simulink model "FOC_sensored"  (R2026a)
settings: Solver=VariableStepAuto  StopTime=0.5  MaxStep=1e-4  RelTol=1e-4
values from neighbouring files (symbols this model uses):
  Encoder_resolution = 4000    [FOC_sensored_script.m]
  In = 1    [FOC_sensored_script.m]
  J = 0.1e-4    (= 1e-05)    [FOC_sensored_script.m]
  Kr_cont_current = (2*omega_n*tau_q*zeta - 1) / K_q    [FOC_sensored_script.m]
  Kr_cont_speed = (2*omega_n_speed*tau_w*zeta_speed - 1) / K_w    [FOC_sensored_script.m]
  Kr_direct_back_current = (1-delta2*exp(Ts_current/tau_q)) / (K_q*(exp(Ts_current/tau_q)-1))    [FOC_sensored_script.m]
  Kr_direct_back_speed = (1-delta2*exp(Ts_speed/tau_w)) / (K_w*(exp(Ts_speed/tau_w)-1))    [FOC_sensored_script.m]
  Kr_direct_forw_current = (1+(1+delta1)*exp(Ts_current/tau_q)) / (K_q*(exp(Ts_current/tau_q)-1))    [FOC_sensored_script.m]
  Kr_direct_tustin_current = (2-exp(Ts_current/tau_q)*(delta2-delta1-1)) / (2*K_q*(exp(Ts_current/tau_q)-1))    [FOC_sensored_script.m]
  Kr_direct_tustin_speed = (2-exp(Ts_speed/tau_w)*(delta2-delta1-1)) / (2*K_w*(exp(Ts_speed/tau_w)-1))    [FOC_sensored_script.m]
  Ls = 330e-6/2    (= 0.000165)    [FOC_sensored_script.m]
  Mn = Pn/wn    [FOC_sensored_script.m]
  nn = ns/pp    (= 6000)    [FOC_sensored_script.m]
  pp = (60*fs)/ns    (= 4)    [FOC_sensored_script.m]
  Psir = 0.0064    [FOC_sensored_script.m]
  T_speed_feedback = 0.0005    [FOC_sensored_script.m]
  Ti_cont_current = (2*omega_n*tau_q*zeta - 1) / (tau_q * omega_n^2)    [FOC_sensored_script.m]
  Ti_cont_speed = (2*omega_n_speed*tau_w*zeta_speed - 1) / (tau_w * omega_n_speed^2)    [FOC_sensored_script.m]
  Ti_direct_back_current = Ts_current * (exp(-Ts_current/tau_q)-delta2) / (1+delta1+delta2)    [FOC_sensored_script.m]
  Ti_direct_back_speed = Ts_speed * (exp(-Ts_speed/tau_w)-delta2) / (1+delta1+delta2)    [FOC_sensored_script.m]
  Ti_direct_forw_current = Ts_current * (1+delta1+exp(-Ts_current/tau_q)) / (1+delta1+delta2)    [FOC_sensored_script.m]
  Ti_direct_forw_speed = Ts_speed * (1+delta1+exp(-Ts_speed/tau_w)) / (1+delta1+delta2)    [FOC_sensored_script.m]
  Ti_direct_tustin_current = Ts_current*(2*exp(-Ts_current/tau_q)+delta1-delta2+1) / (2*(1+delta1+delta2))    [FOC_sensored_script.m]
  Ti_direct_tustin_speed = Ts_speed*(2*exp(-Ts_speed/tau_w)+delta1-delta2+1) / (2*(1+delta1+delta2))    [FOC_sensored_script.m]
  Ts_current = 100e-6    (= 0.0001)    [FOC_sensored_script.m]
  Udc = 24    [FOC_sensored_script.m]
undefined symbols (not defined in the file or in its folder): Ld, Lq
libraries: fl_lib x48, nesl_utility x42, ee_lib x18, eeTransforms x12
(part 1 of 3)
settings Model: Creator=LukaPravica  LastModifiedBy=Rio
settings SimscapeCC: ExplicitSolverDiagnosticOptions=none  SimscapeNominalValues="[{\"value\":\"1\",\"unit\":\"A\"},{\"value\":\"1\",\"unit\":\"bar\"},{\"value\":\"1\",\"unit\":\"cm^2\"},{\"value\":\"1\",\"unit\":\"cm^3/s\"},{\"value\":\"1\",\"unit\":\"kJ/kg\"},{\"value\":\"1\",\"unit\":\"kW\"},{\"value\":\"1\",\"unit\":\"l\"},{\"value\":\"1\",\"unit\":\"N\"},{\"value\":\"1\",\"unit\":\"N*m\"},{\"value\":\"1\",\"unit\":\"V\"}]"  SimscapeLogType=none  SimscapeLogDataHistory=5000.0

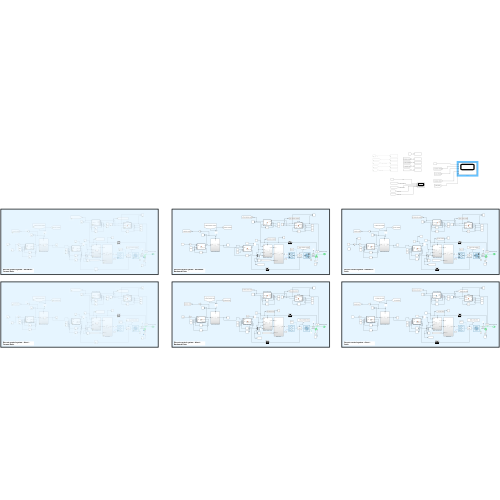
[thumbnail: Simulink's stored preview of the top-level diagram]
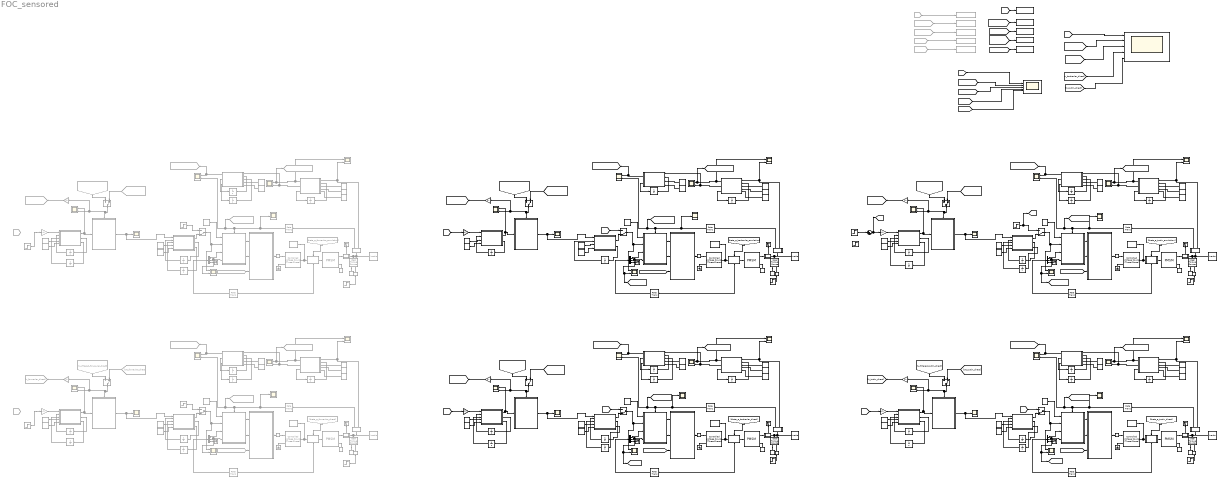
== system FOC_sensored ==
  note: Discrete control system - emulation - Tustin
  note: Discrete control system - direct - Tustin
  note: Discrete control system - emulation -
      | Backward Euler
  note: Discrete control system - direct - Backward Euler
  note: Discrete control system - emulation -
      | Forward Euler
  note: Discrete control system - direct -
      | Forward Euler
  Constant{,1,20,30} (4 alike) : Constant  Value=0  SampleTime=Ts_current
  Constant{3,5,8,10..11,13,15,18,21,23,25,28,31,33,35,38} (16 alike) : Constant  Value=Ts_current  SampleTime=Ts_current
  Constant{2,12,22,32} (4 alike) : Constant  Value=1/(2*pi*T_speed_feedback)  SampleTime=Ts_current
  Constant{4,14,24,34} (4 alike) : Constant  Value=Encoder_resolution  SampleTime=Ts_current
  Constant{6,16,26,36} (4 alike) : Constant  Value=pp  SampleTime=Ts_current
  Constant17 : Constant  Value=1/(2*pi*Ti_direct_tustin_current)  SampleTime=Ts_current
  Constant19 : Constant  Value=1/(2*pi*Ti_direct_tustin_speed)  SampleTime=Ts_current
  Constant27 : Constant  Value=1/(2*pi*Ti_cont_current)  SampleTime=Ts_current
  Constant29 : Constant  Value=1/(2*pi*Ti_cont_speed)  SampleTime=Ts_current
  Constant37 : Constant  Value=1/(2*pi*Ti_direct_back_current)  SampleTime=Ts_current
  Constant39 : Constant  Value=1/(2*pi*Ti_direct_back_speed)  SampleTime=Ts_current
  Constant40 : Constant  Commented=on  Value=0  SampleTime=Ts_current
  Constant{41,43,45,48,51,53,55,58} (8 alike) : Constant  Commented=on  Value=Ts_current  SampleTime=Ts_current
  Constant42 : Constant  Commented=on  Value=1/(2*pi*T_speed_feedback)  SampleTime=Ts_current
  Constant44 : Constant  Commented=on  Value=Encoder_resolution  SampleTime=Ts_current
  Constant46 : Constant  Commented=on  Value=pp  SampleTime=Ts_current
  Constant47 : Constant  Commented=on  Value=1/(2*pi*Ti_cont_current)  SampleTime=Ts_current
  Constant49 : Constant  Commented=on  Value=1/(2*pi*Ti_cont_speed)  SampleTime=Ts_current
  Constant50 : Constant  Commented=on  Value=0  SampleTime=Ts_current
  Constant52 : Constant  Commented=on  Value=1/(2*pi*T_speed_feedback)  SampleTime=Ts_current
  Constant54 : Constant  Commented=on  Value=Encoder_resolution  SampleTime=Ts_current
  Constant56 : Constant  Commented=on  Value=pp  SampleTime=Ts_current
  Constant57 : Constant  Commented=on  Value=1/(2*pi*Ti_direct_forw_current)  SampleTime=Ts_current
  Constant59 : Constant  Commented=on  Value=1/(2*pi*Ti_direct_forw_speed)  SampleTime=Ts_current
  Constant7 : Constant  Value=1/(2*pi*Ti_cont_current)  SampleTime=Ts_current
  Constant9 : Constant  Value=1/(2*pi*Ti_cont_speed)  SampleTime=Ts_current
  Controlled Voltage Source (Three-Phase){1,3..4,7} (4 alike) : ee_lib/Sources/Controlled Voltage Source (Three-Phase)  input_option=ee.enum.inputType.instantaneous  FRated=60 Hz
  Controlled Voltage Source (Three-Phase)2 : ee_lib/Sources/Controlled Voltage Source (Three-Phase)  Commented=on  input_option=ee.enum.inputType.instantaneous  FRated=60 Hz
  Controlled Voltage Source (Three-Phase)5 : ee_lib/Sources/Controlled Voltage Source (Three-Phase)  Commented=on  input_option=ee.enum.inputType.instantaneous  FRated=60 Hz
  Demux{1,3..4,7} (4 alike) : Demux  Outputs=3
  Demux2 : Demux  Commented=on  Outputs=3
  Demux5 : Demux  Commented=on  Outputs=3
  Diskretni regulator brzine1 : Subsystem
      settings: PortSchema="{\"entries\":[{\"content\":{\"sides\":[{\"content\":{\"connectorIds\":[\"In1\"]},\"type\":\"ConnectorPlacement.EquallySpacedRectSide\",\"uuid\":\"a9765fbc-5a4d-474e-be8d-5c320c5f07ca\"},{\"content\":{\"connectorIds\":[\"Out1\"],\"side\":\"RIGHT\"},\"type\":\"ConnectorPlacement.EquallySpacedRectSide\",\"uuid\":\"d113e0d0-4772-4877-8676-69342ee8f64f\"},{\"content\":{\"connectorIds\":[\"In2\"],\"side\":\"TOP\"},\"type\":\"ConnectorPlacement.EquallySpacedRectSide\",\"uuid\":\"4ca0dc59-fd41-4846-82a7-6904cf53659d\"}]},\"type\":\"ConnectorPlacement.EquallySpacedConnector\",\"uuid\":\"7fdfac1a-ebdc-43ed-9adb-be729266989d\"}],\"packageUris\":[\"http://schema.mathworks.com/mf0/Connector/R2020b\"],\"version\":\"1.0\"}"
  Diskretni regulator brzine2 : Subsystem
      settings: PortSchema="{\"entries\":[{\"content\":{\"sides\":[{\"content\":{\"connectorIds\":[\"In1\"]},\"type\":\"ConnectorPlacement.EquallySpacedRectSide\",\"uuid\":\"a9765fbc-5a4d-474e-be8d-5c320c5f07ca\"},{\"content\":{\"connectorIds\":[\"Out1\"],\"side\":\"RIGHT\"},\"type\":\"ConnectorPlacement.EquallySpacedRectSide\",\"uuid\":\"d113e0d0-4772-4877-8676-69342ee8f64f\"},{\"content\":{\"connectorIds\":[\"In2\"],\"side\":\"TOP\"},\"type\":\"ConnectorPlacement.EquallySpacedRectSide\",\"uuid\":\"4ca0dc59-fd41-4846-82a7-6904cf53659d\"}]},\"type\":\"ConnectorPlacement.EquallySpacedConnector\",\"uuid\":\"7fdfac1a-ebdc-43ed-9adb-be729266989d\"}],\"packageUris\":[\"http://schema.mathworks.com/mf0/Connector/R2020b\"],\"version\":\"1.0\"}"
  Diskretni regulator brzine3 : Subsystem
      settings: PortSchema="{\"entries\":[{\"content\":{\"sides\":[{\"content\":{\"connectorIds\":[\"In1\"]},\"type\":\"ConnectorPlacement.EquallySpacedRectSide\",\"uuid\":\"a9765fbc-5a4d-474e-be8d-5c320c5f07ca\"},{\"content\":{\"connectorIds\":[\"Out1\"],\"side\":\"RIGHT\"},\"type\":\"ConnectorPlacement.EquallySpacedRectSide\",\"uuid\":\"d113e0d0-4772-4877-8676-69342ee8f64f\"},{\"content\":{\"connectorIds\":[\"In2\"],\"side\":\"TOP\"},\"type\":\"ConnectorPlacement.EquallySpacedRectSide\",\"uuid\":\"4ca0dc59-fd41-4846-82a7-6904cf53659d\"}]},\"type\":\"ConnectorPlacement.EquallySpacedConnector\",\"uuid\":\"7fdfac1a-ebdc-43ed-9adb-be729266989d\"}],\"packageUris\":[\"http://schema.mathworks.com/mf0/Connector/R2020b\"],\"version\":\"1.0\"}"
  Diskretni regulator brzine4 : Subsystem  Commented=on
      settings: PortSchema="{\"entries\":[{\"content\":{\"sides\":[{\"content\":{\"connectorIds\":[\"In1\"]},\"type\":\"ConnectorPlacement.EquallySpacedRectSide\",\"uuid\":\"a9765fbc-5a4d-474e-be8d-5c320c5f07ca\"},{\"content\":{\"connectorIds\":[\"Out1\"],\"side\":\"RIGHT\"},\"type\":\"ConnectorPlacement.EquallySpacedRectSide\",\"uuid\":\"d113e0d0-4772-4877-8676-69342ee8f64f\"},{\"content\":{\"connectorIds\":[\"In2\"],\"side\":\"TOP\"},\"type\":\"ConnectorPlacement.EquallySpacedRectSide\",\"uuid\":\"4ca0dc59-fd41-4846-82a7-6904cf53659d\"}]},\"type\":\"ConnectorPlacement.EquallySpacedConnector\",\"uuid\":\"7fdfac1a-ebdc-43ed-9adb-be729266989d\"}],\"packageUris\":[\"http://schema.mathworks.com/mf0/Connector/R2020b\"],\"version\":\"1.0\"}"
  Diskretni regulator brzine5 : Subsystem
      settings: PortSchema="{\"entries\":[{\"content\":{\"sides\":[{\"content\":{\"connectorIds\":[\"In1\"]},\"type\":\"ConnectorPlacement.EquallySpacedRectSide\",\"uuid\":\"a9765fbc-5a4d-474e-be8d-5c320c5f07ca\"},{\"content\":{\"connectorIds\":[\"Out1\"],\"side\":\"RIGHT\"},\"type\":\"ConnectorPlacement.EquallySpacedRectSide\",\"uuid\":\"d113e0d0-4772-4877-8676-69342ee8f64f\"},{\"content\":{\"connectorIds\":[\"In2\"],\"side\":\"TOP\"},\"type\":\"ConnectorPlacement.EquallySpacedRectSide\",\"uuid\":\"4ca0dc59-fd41-4846-82a7-6904cf53659d\"}]},\"type\":\"ConnectorPlacement.EquallySpacedConnector\",\"uuid\":\"7fdfac1a-ebdc-43ed-9adb-be729266989d\"}],\"packageUris\":[\"http://schema.mathworks.com/mf0/Connector/R2020b\"],\"version\":\"1.0\"}"
  Diskretni regulator brzine6 : Subsystem  Commented=on
      settings: PortSchema="{\"entries\":[{\"content\":{\"sides\":[{\"content\":{\"connectorIds\":[\"In1\"]},\"type\":\"ConnectorPlacement.EquallySpacedRectSide\",\"uuid\":\"a9765fbc-5a4d-474e-be8d-5c320c5f07ca\"},{\"content\":{\"connectorIds\":[\"Out1\"],\"side\":\"RIGHT\"},\"type\":\"ConnectorPlacement.EquallySpacedRectSide\",\"uuid\":\"d113e0d0-4772-4877-8676-69342ee8f64f\"},{\"content\":{\"connectorIds\":[\"In2\"],\"side\":\"TOP\"},\"type\":\"ConnectorPlacement.EquallySpacedRectSide\",\"uuid\":\"4ca0dc59-fd41-4846-82a7-6904cf53659d\"}]},\"type\":\"ConnectorPlacement.EquallySpacedConnector\",\"uuid\":\"7fdfac1a-ebdc-43ed-9adb-be729266989d\"}],\"packageUris\":[\"http://schema.mathworks.com/mf0/Connector/R2020b\"],\"version\":\"1.0\"}"
  Diskretni regulatori struje1 : Subsystem
      settings: PortSchema="{\"entries\":[{\"content\":{\"sides\":[{\"content\":{\"connectorIds\":[\"In1\",\"In2\",\"In3\",\"In4\"]},\"type\":\"ConnectorPlacement.EquallySpacedRectSide\",\"uuid\":\"d3a62493-f7c6-444f-9476-25937989f6ea\"},{\"content\":{\"connectorIds\":[\"Out1\",\"Out2\"],\"side\":\"RIGHT\"},\"type\":\"ConnectorPlacement.EquallySpacedRectSide\",\"uuid\":\"ca5c9823-b9be-4b72-ab87-a2cad855a0f6\"},{\"content\":{\"connectorIds\":[\"In5\"],\"side\":\"TOP\"},\"type\":\"ConnectorPlacement.EquallySpacedRectSide\",\"uuid\":\"496b345e-fed9-4adb-95d9-010d07f11d94\"}]},\"type\":\"ConnectorPlacement.EquallySpacedConnector\",\"uuid\":\"9eb14200-6fae-48ad-9447-ab4bb77ea536\"}],\"packageUris\":[\"http://schema.mathworks.com/mf0/Connector/R2020b\"],\"version\":\"1.0\"}"
  Diskretni regulatori struje2 : Subsystem
      settings: PortSchema="{\"entries\":[{\"content\":{\"sides\":[{\"content\":{\"connectorIds\":[\"In1\",\"In2\",\"In3\",\"In4\"]},\"type\":\"ConnectorPlacement.EquallySpacedRectSide\",\"uuid\":\"d3a62493-f7c6-444f-9476-25937989f6ea\"},{\"content\":{\"connectorIds\":[\"Out1\",\"Out2\"],\"side\":\"RIGHT\"},\"type\":\"ConnectorPlacement.EquallySpacedRectSide\",\"uuid\":\"ca5c9823-b9be-4b72-ab87-a2cad855a0f6\"},{\"content\":{\"connectorIds\":[\"In5\"],\"side\":\"TOP\"},\"type\":\"ConnectorPlacement.EquallySpacedRectSide\",\"uuid\":\"496b345e-fed9-4adb-95d9-010d07f11d94\"}]},\"type\":\"ConnectorPlacement.EquallySpacedConnector\",\"uuid\":\"9eb14200-6fae-48ad-9447-ab4bb77ea536\"}],\"packageUris\":[\"http://schema.mathworks.com/mf0/Connector/R2020b\"],\"version\":\"1.0\"}"
  Diskretni regulatori struje3 : Subsystem
      settings: PortSchema="{\"entries\":[{\"content\":{\"sides\":[{\"content\":{\"connectorIds\":[\"In1\",\"In2\",\"In3\",\"In4\"]},\"type\":\"ConnectorPlacement.EquallySpacedRectSide\",\"uuid\":\"d3a62493-f7c6-444f-9476-25937989f6ea\"},{\"content\":{\"connectorIds\":[\"Out1\",\"Out2\"],\"side\":\"RIGHT\"},\"type\":\"ConnectorPlacement.EquallySpacedRectSide\",\"uuid\":\"ca5c9823-b9be-4b72-ab87-a2cad855a0f6\"},{\"content\":{\"connectorIds\":[\"In5\"],\"side\":\"TOP\"},\"type\":\"ConnectorPlacement.EquallySpacedRectSide\",\"uuid\":\"496b345e-fed9-4adb-95d9-010d07f11d94\"}]},\"type\":\"ConnectorPlacement.EquallySpacedConnector\",\"uuid\":\"9eb14200-6fae-48ad-9447-ab4bb77ea536\"}],\"packageUris\":[\"http://schema.mathworks.com/mf0/Connector/R2020b\"],\"version\":\"1.0\"}"
  Diskretni regulatori struje4 : Subsystem  Commented=on
      settings: PortSchema="{\"entries\":[{\"content\":{\"sides\":[{\"content\":{\"connectorIds\":[\"In1\",\"In2\",\"In3\",\"In4\"]},\"type\":\"ConnectorPlacement.EquallySpacedRectSide\",\"uuid\":\"d3a62493-f7c6-444f-9476-25937989f6ea\"},{\"content\":{\"connectorIds\":[\"Out1\",\"Out2\"],\"side\":\"RIGHT\"},\"type\":\"ConnectorPlacement.EquallySpacedRectSide\",\"uuid\":\"ca5c9823-b9be-4b72-ab87-a2cad855a0f6\"},{\"content\":{\"connectorIds\":[\"In5\"],\"side\":\"TOP\"},\"type\":\"ConnectorPlacement.EquallySpacedRectSide\",\"uuid\":\"496b345e-fed9-4adb-95d9-010d07f11d94\"}]},\"type\":\"ConnectorPlacement.EquallySpacedConnector\",\"uuid\":\"9eb14200-6fae-48ad-9447-ab4bb77ea536\"}],\"packageUris\":[\"http://schema.mathworks.com/mf0/Connector/R2020b\"],\"version\":\"1.0\"}"
  Diskretni regulatori struje5 : Subsystem
      settings: PortSchema="{\"entries\":[{\"content\":{\"sides\":[{\"content\":{\"connectorIds\":[\"In1\",\"In2\",\"In3\",\"In4\"]},\"type\":\"ConnectorPlacement.EquallySpacedRectSide\",\"uuid\":\"d3a62493-f7c6-444f-9476-25937989f6ea\"},{\"content\":{\"connectorIds\":[\"Out1\",\"Out2\"],\"side\":\"RIGHT\"},\"type\":\"ConnectorPlacement.EquallySpacedRectSide\",\"uuid\":\"ca5c9823-b9be-4b72-ab87-a2cad855a0f6\"},{\"content\":{\"connectorIds\":[\"In5\"],\"side\":\"TOP\"},\"type\":\"ConnectorPlacement.EquallySpacedRectSide\",\"uuid\":\"496b345e-fed9-4adb-95d9-010d07f11d94\"}]},\"type\":\"ConnectorPlacement.EquallySpacedConnector\",\"uuid\":\"9eb14200-6fae-48ad-9447-ab4bb77ea536\"}],\"packageUris\":[\"http://schema.mathworks.com/mf0/Connector/R2020b\"],\"version\":\"1.0\"}"
  Diskretni regulatori struje6 : Subsystem  Commented=on
      settings: PortSchema="{\"entries\":[{\"content\":{\"sides\":[{\"content\":{\"connectorIds\":[\"In1\",\"In2\",\"In3\",\"In4\"]},\"type\":\"ConnectorPlacement.EquallySpacedRectSide\",\"uuid\":\"d3a62493-f7c6-444f-9476-25937989f6ea\"},{\"content\":{\"connectorIds\":[\"Out1\",\"Out2\"],\"side\":\"RIGHT\"},\"type\":\"ConnectorPlacement.EquallySpacedRectSide\",\"uuid\":\"ca5c9823-b9be-4b72-ab87-a2cad855a0f6\"},{\"content\":{\"connectorIds\":[\"In5\"],\"side\":\"TOP\"},\"type\":\"ConnectorPlacement.EquallySpacedRectSide\",\"uuid\":\"496b345e-fed9-4adb-95d9-010d07f11d94\"}]},\"type\":\"ConnectorPlacement.EquallySpacedConnector\",\"uuid\":\"9eb14200-6fae-48ad-9447-ab4bb77ea536\"}],\"packageUris\":[\"http://schema.mathworks.com/mf0/Connector/R2020b\"],\"version\":\"1.0\"}"
  Electrical Reference{1..3,6} (4 alike) : fl_lib/Electrical/Electrical Elements/Electrical Reference
  Electrical Reference4 : fl_lib/Electrical/Electrical Elements/Electrical Reference  Commented=on
  Electrical Reference5 : fl_lib/Electrical/Electrical Elements/Electrical Reference  Commented=on
  Encoder : MATLAB Function  TreatAsAtomicUnit=on
  Encoder1 : MATLAB Function  TreatAsAtomicUnit=on
  Encoder2 : MATLAB Function  TreatAsAtomicUnit=on
  Encoder3 : MATLAB Function  TreatAsAtomicUnit=on
  Encoder4 : MATLAB Function  Commented=on  TreatAsAtomicUnit=on
  Encoder5 : MATLAB Function  Commented=on  TreatAsAtomicUnit=on
  From32 : From  Commented=on  GotoTag=theta_e_forweuler_emulation
  From33 : From  Commented=on  GotoTag=w_filtered_forweuler_emulation
  From34 : From  Commented=on  GotoTag=theta_e_forweuler_emulation
  From35 : From  Commented=on  GotoTag=we_forweuler_emulation
  From36 : From  Commented=on  GotoTag=n_ref
  From38 : From  Commented=on  GotoTag=theta_e_forweuler_direct
  From39 : From  Commented=on  GotoTag=w_filtered_forweuler_direct
  From40 : From  Commented=on  GotoTag=theta_e_forweuler_direct
  From41 : From  Commented=on  GotoTag=we_forweuler_direct
  From42 : From  Commented=on  GotoTag=n_ref
  From46 : From  Commented=on  GotoTag=i_disc_emu_back
  From47 : From  Commented=on  GotoTag=i_disc_emu_tustin
  From48 : From  Commented=on  GotoTag=i_direct_back
  From49 : From  Commented=on  GotoTag=i_direct_tustin
  From50 : From  Commented=on  GotoTag=i_ref
  Gain{1,3,5,7} (4 alike) : Gain  Gain=pp*pi/30
  Gain{2,4,6,15} (4 alike) : Gain  Gain=30/pi/pp
  Gain16 : Gain  Commented=on  Gain=pp*pi/30
  Gain17 : Gain  Commented=on  Gain=30/pi/pp
  Gain18 : Gain  Commented=on  Gain=pp*pi/30
  Gain19 : Gain  Commented=on  Gain=30/pi/pp
  Goto18 : Goto  Commented=on  GotoTag=w_filtered_forweuler_emulation
  Goto19 : Goto  Commented=on  GotoTag=we_forweuler_emulation
  Goto20 : Goto  Commented=on  GotoTag=n_forweuler_emulation
  Goto21 : Goto  Commented=on  GotoTag=theta_e_forweuler_emulation
  Goto22 : Goto  Commented=on  GotoTag=w_filtered_forweuler_direct
  Goto23 : Goto  Commented=on  GotoTag=we_forweuler_direct
  Goto24 : Goto  Commented=on  GotoTag=n_forweuler_direct
  Goto25 : Goto  Commented=on  GotoTag=theta_e_forweuler_direct
  Ideal Torque Source{1,3..4,7} (4 alike) : fl_lib/Mechanical/Mechanical Sources/Ideal Torque Source
  Ideal Torque Source2 : fl_lib/Mechanical/Mechanical Sources/Ideal Torque Source  Commented=on
  Ideal Torque Source5 : fl_lib/Mechanical/Mechanical Sources/Ideal Torque Source  Commented=on
  Inertia{,1..3} (4 alike) : fl_lib/Mechanical/Rotational Elements/Inertia  inertia=J kg*m^2  num_ports=foundation.enum.numPorts2.one  w_specify=off  w_priority=High  w=0 rad/s  w_nominal_specify=off  w_nominal_value=1  w_nominal_unit=rad/s  t_specify=off  t_priority=None  t=0 N*m  t_nominal_specify=off  t_nominal_value=1  t_nominal_unit=N*m
  Inertia4 : fl_lib/Mechanical/Rotational Elements/Inertia  Commented=on  inertia=J kg*m^2  num_ports=foundation.enum.numPorts2.one  w_specify=off  w_priority=High  w=0 rad/s  w_nominal_specify=off  w_nominal_value=1  w_nominal_unit=rad/s  t_specify=off  t_priority=None  t=0 N*m  t_nominal_specify=off  t_nominal_value=1  t_nominal_unit=N*m
  Inertia5 : fl_lib/Mechanical/Rotational Elements/Inertia  Commented=on  inertia=J kg*m^2  num_ports=foundation.enum.numPorts2.one  w_specify=off  w_priority=High  w=0 rad/s  w_nominal_specify=off  w_nominal_value=1  w_nominal_unit=rad/s  t_specify=off  t_priority=None  t=0 N*m  t_nominal_specify=off  t_nominal_value=1  t_nominal_unit=N*m
  Low-Pass Filter Current : MATLAB Function  TreatAsAtomicUnit=on
  Low-Pass Filter Current1 : MATLAB Function  TreatAsAtomicUnit=on
  Low-Pass Filter Current2 : MATLAB Function  TreatAsAtomicUnit=on
  Low-Pass Filter Current3 : MATLAB Function  TreatAsAtomicUnit=on
  Low-Pass Filter Current4 : MATLAB Function  Commented=on  TreatAsAtomicUnit=on
  Low-Pass Filter Current5 : MATLAB Function  Commented=on  TreatAsAtomicUnit=on
  Low-Pass Filter Speed : MATLAB Function  TreatAsAtomicUnit=on
  Low-Pass Filter Speed Ref : MATLAB Function  TreatAsAtomicUnit=on
  Low-Pass Filter Speed Ref1 : MATLAB Function  TreatAsAtomicUnit=on
  Low-Pass Filter Speed Ref2 : MATLAB Function  TreatAsAtomicUnit=on
  Low-Pass Filter Speed Ref3 : MATLAB Function  TreatAsAtomicUnit=on
  Low-Pass Filter Speed Ref4 : MATLAB Function  Commented=on  TreatAsAtomicUnit=on
  Low-Pass Filter Speed Ref5 : MATLAB Function  Commented=on  TreatAsAtomicUnit=on
  Low-Pass Filter Speed1 : MATLAB Function  TreatAsAtomicUnit=on
  Low-Pass Filter Speed2 : MATLAB Function  TreatAsAtomicUnit=on
  Low-Pass Filter Speed3 : MATLAB Function  TreatAsAtomicUnit=on
  Low-Pass Filter Speed4 : MATLAB Function  Commented=on  TreatAsAtomicUnit=on
  Low-Pass Filter Speed5 : MATLAB Function  Commented=on  TreatAsAtomicUnit=on
  Manual Switch{,1..7} (8 alike) : ManualSwitch  CurrentSetting=0
  Manual Switch{8..11} (4 alike) : ManualSwitch  Commented=on  CurrentSetting=0
  Mechanical Rotational Reference{1..6,11..12} (8 alike) : fl_lib/Mechanical/Rotational Elements/Mechanical Rotational Reference
  Mechanical Rotational Reference{7..10} (4 alike) : fl_lib/Mechanical/Rotational Elements/Mechanical Rotational Reference  Commented=on
  Mjerenje momenta1 : Subsystem
      settings: PortSchema="{\"entries\":[{\"content\":{\"sides\":[{\"content\":{\"connectorIds\":[\"LConn1\"]},\"type\":\"ConnectorPlacement.EquallySpacedRectSide\",\"uuid\":\"6fa7c16c-6de5-49c8-bc22-739ef8014510\"},{\"content\":{\"connectorIds\":[\"RConn1\"],\"side\":\"RIGHT\"},\"type\":\"ConnectorPlacement.EquallySpacedRectSide\",\"uuid\":\"6cbb3fe1-95dc-4f03-932b-ab8cb637a208\"},{\"content\":{\"connectorIds\":[\"Out1\"],\"side\":\"TOP\"},\"type\":\"ConnectorPlacement.EquallySpacedRectSide\",\"uuid\":\"35a7ae71-901f-47d3-ac0b-d21c2464290d\"}]},\"type\":\"ConnectorPlacement.EquallySpacedConnector\",\"uuid\":\"03aa7740-1fdb-47bb-9a21-844669f6bcda\"}],\"packageUris\":[\"http://schema.mathworks.com/mf0/Connector/R2020b\"],\"version\":\"1.0\"}"
      mask Display: disp('trq')
  Mjerenje momenta2 : Subsystem
      settings: PortSchema="{\"entries\":[{\"content\":{\"sides\":[{\"content\":{\"connectorIds\":[\"LConn1\"]},\"type\":\"ConnectorPlacement.EquallySpacedRectSide\",\"uuid\":\"6fa7c16c-6de5-49c8-bc22-739ef8014510\"},{\"content\":{\"connectorIds\":[\"RConn1\"],\"side\":\"RIGHT\"},\"type\":\"ConnectorPlacement.EquallySpacedRectSide\",\"uuid\":\"6cbb3fe1-95dc-4f03-932b-ab8cb637a208\"},{\"content\":{\"connectorIds\":[\"Out1\"],\"side\":\"TOP\"},\"type\":\"ConnectorPlacement.EquallySpacedRectSide\",\"uuid\":\"35a7ae71-901f-47d3-ac0b-d21c2464290d\"}]},\"type\":\"ConnectorPlacement.EquallySpacedConnector\",\"uuid\":\"03aa7740-1fdb-47bb-9a21-844669f6bcda\"}],\"packageUris\":[\"http://schema.mathworks.com/mf0/Connector/R2020b\"],\"version\":\"1.0\"}"
      mask Display: disp('trq')
  Mjerenje momenta3 : Subsystem
      settings: PortSchema="{\"entries\":[{\"content\":{\"sides\":[{\"content\":{\"connectorIds\":[\"LConn1\"]},\"type\":\"ConnectorPlacement.EquallySpacedRectSide\",\"uuid\":\"6fa7c16c-6de5-49c8-bc22-739ef8014510\"},{\"content\":{\"connectorIds\":[\"RConn1\"],\"side\":\"RIGHT\"},\"type\":\"ConnectorPlacement.EquallySpacedRectSide\",\"uuid\":\"6cbb3fe1-95dc-4f03-932b-ab8cb637a208\"},{\"content\":{\"connectorIds\":[\"Out1\"],\"side\":\"TOP\"},\"type\":\"ConnectorPlacement.EquallySpacedRectSide\",\"uuid\":\"35a7ae71-901f-47d3-ac0b-d21c2464290d\"}]},\"type\":\"ConnectorPlacement.EquallySpacedConnector\",\"uuid\":\"03aa7740-1fdb-47bb-9a21-844669f6bcda\"}],\"packageUris\":[\"http://schema.mathworks.com/mf0/Connector/R2020b\"],\"version\":\"1.0\"}"
      mask Display: disp('trq')
  Mjerenje momenta4 : Subsystem  Commented=on
      settings: PortSchema="{\"entries\":[{\"content\":{\"sides\":[{\"content\":{\"connectorIds\":[\"LConn1\"]},\"type\":\"ConnectorPlacement.EquallySpacedRectSide\",\"uuid\":\"6fa7c16c-6de5-49c8-bc22-739ef8014510\"},{\"content\":{\"connectorIds\":[\"RConn1\"],\"side\":\"RIGHT\"},\"type\":\"ConnectorPlacement.EquallySpacedRectSide\",\"uuid\":\"6cbb3fe1-95dc-4f03-932b-ab8cb637a208\"},{\"content\":{\"connectorIds\":[\"Out1\"],\"side\":\"TOP\"},\"type\":\"ConnectorPlacement.EquallySpacedRectSide\",\"uuid\":\"35a7ae71-901f-47d3-ac0b-d21c2464290d\"}]},\"type\":\"ConnectorPlacement.EquallySpacedConnector\",\"uuid\":\"03aa7740-1fdb-47bb-9a21-844669f6bcda\"}],\"packageUris\":[\"http://schema.mathworks.com/mf0/Connector/R2020b\"],\"version\":\"1.0\"}"
      mask Display: disp('trq')
  Mjerenje momenta5 : Subsystem  Commented=on
      settings: PortSchema="{\"entries\":[{\"content\":{\"sides\":[{\"content\":{\"connectorIds\":[\"LConn1\"]},\"type\":\"ConnectorPlacement.EquallySpacedRectSide\",\"uuid\":\"6fa7c16c-6de5-49c8-bc22-739ef8014510\"},{\"content\":{\"connectorIds\":[\"RConn1\"],\"side\":\"RIGHT\"},\"type\":\"ConnectorPlacement.EquallySpacedRectSide\",\"uuid\":\"6cbb3fe1-95dc-4f03-932b-ab8cb637a208\"},{\"content\":{\"connectorIds\":[\"Out1\"],\"side\":\"TOP\"},\"type\":\"ConnectorPlacement.EquallySpacedRectSide\",\"uuid\":\"35a7ae71-901f-47d3-ac0b-d21c2464290d\"}]},\"type\":\"ConnectorPlacement.EquallySpacedConnector\",\"uuid\":\"03aa7740-1fdb-47bb-9a21-844669f6bcda\"}],\"packageUris\":[\"http://schema.mathworks.com/mf0/Connector/R2020b\"],\"version\":\"1.0\"}"
      mask Display: disp('trq')
  Mjerenje momenta6 : Subsystem
      settings: PortSchema="{\"entries\":[{\"content\":{\"sides\":[{\"content\":{\"connectorIds\":[\"LConn1\"]},\"type\":\"ConnectorPlacement.EquallySpacedRectSide\",\"uuid\":\"6fa7c16c-6de5-49c8-bc22-739ef8014510\"},{\"content\":{\"connectorIds\":[\"RConn1\"],\"side\":\"RIGHT\"},\"type\":\"ConnectorPlacement.EquallySpacedRectSide\",\"uuid\":\"6cbb3fe1-95dc-4f03-932b-ab8cb637a208\"},{\"content\":{\"connectorIds\":[\"Out1\"],\"side\":\"TOP\"},\"type\":\"ConnectorPlacement.EquallySpacedRectSide\",\"uuid\":\"35a7ae71-901f-47d3-ac0b-d21c2464290d\"}]},\"type\":\"ConnectorPlacement.EquallySpacedConnector\",\"uuid\":\"03aa7740-1fdb-47bb-9a21-844669f6bcda\"}],\"packageUris\":[\"http://schema.mathworks.com/mf0/Connector/R2020b\"],\"version\":\"1.0\"}"
      mask Display: disp('trq')
  Mjerenje kuta i brzine1 : Subsystem
      mask Display: disp('w,a')
  Mjerenje kuta i brzine2 : Subsystem
      mask Display: disp('w,a')
  Mjerenje kuta i brzine3 : Subsystem
      mask Display: disp('w,a')
  Mjerenje kuta i brzine4 : Subsystem  Commented=on
      mask Display: disp('w,a')
  Mjerenje kuta i brzine5 : Subsystem  Commented=on
      mask Display: disp('w,a')
  Mjerenje kuta i brzine6 : Subsystem
      mask Display: disp('w,a')
  Mjerenje struje1 : Subsystem
      settings: PortSchema="{\"entries\":[{\"content\":{\"sides\":[{\"content\":{\"connectorIds\":[\"LConn1\"]},\"type\":\"ConnectorPlacement.EquallySpacedRectSide\",\"uuid\":\"6fa7c16c-6de5-49c8-bc22-739ef8014510\"},{\"content\":{\"connectorIds\":[\"RConn1\"],\"side\":\"RIGHT\"},\"type\":\"ConnectorPlacement.EquallySpacedRectSide\",\"uuid\":\"6cbb3fe1-95dc-4f03-932b-ab8cb637a208\"},{\"content\":{\"connectorIds\":[\"In1\"],\"side\":\"TOP\"},\"type\":\"ConnectorPlacement.EquallySpacedRectSide\",\"uuid\":\"35a7ae71-901f-47d3-ac0b-d21c2464290d\"},{\"content\":{\"connectorIds\":[\"Out1\"],\"side\":\"BOTTOM\"},\"type\":\"ConnectorPlacement.EquallySpacedRectSide\",\"uuid\":\"976aabfd-697c-47ce-8be7-acff7370fc8c\"}]},\"type\":\"ConnectorPlacement.EquallySpacedConnector\",\"uuid\":\"03aa7740-1fdb-47bb-9a21-844669f6bcda\"}],\"packageUris\":[\"http://schema.mathworks.com/mf0/Connector/R2020b\"],\"version\":\"1.0\"}"
      mask Display: disp('vi abc')
  Mjerenje struje2 : Subsystem
      settings: PortSchema="{\"entries\":[{\"content\":{\"sides\":[{\"content\":{\"connectorIds\":[\"LConn1\"]},\"type\":\"ConnectorPlacement.EquallySpacedRectSide\",\"uuid\":\"6fa7c16c-6de5-49c8-bc22-739ef8014510\"},{\"content\":{\"connectorIds\":[\"RConn1\"],\"side\":\"RIGHT\"},\"type\":\"ConnectorPlacement.EquallySpacedRectSide\",\"uuid\":\"6cbb3fe1-95dc-4f03-932b-ab8cb637a208\"},{\"content\":{\"connectorIds\":[\"In1\"],\"side\":\"TOP\"},\"type\":\"ConnectorPlacement.EquallySpacedRectSide\",\"uuid\":\"35a7ae71-901f-47d3-ac0b-d21c2464290d\"},{\"content\":{\"connectorIds\":[\"Out1\"],\"side\":\"BOTTOM\"},\"type\":\"ConnectorPlacement.EquallySpacedRectSide\",\"uuid\":\"976aabfd-697c-47ce-8be7-acff7370fc8c\"}]},\"type\":\"ConnectorPlacement.EquallySpacedConnector\",\"uuid\":\"03aa7740-1fdb-47bb-9a21-844669f6bcda\"}],\"packageUris\":[\"http://schema.mathworks.com/mf0/Connector/R2020b\"],\"version\":\"1.0\"}"
      mask Display: disp('vi abc')
  Mjerenje struje3 : Subsystem
      settings: PortSchema="{\"entries\":[{\"content\":{\"sides\":[{\"content\":{\"connectorIds\":[\"LConn1\"]},\"type\":\"ConnectorPlacement.EquallySpacedRectSide\",\"uuid\":\"6fa7c16c-6de5-49c8-bc22-739ef8014510\"},{\"content\":{\"connectorIds\":[\"RConn1\"],\"side\":\"RIGHT\"},\"type\":\"ConnectorPlacement.EquallySpacedRectSide\",\"uuid\":\"6cbb3fe1-95dc-4f03-932b-ab8cb637a208\"},{\"content\":{\"connectorIds\":[\"In1\"],\"side\":\"TOP\"},\"type\":\"ConnectorPlacement.EquallySpacedRectSide\",\"uuid\":\"35a7ae71-901f-47d3-ac0b-d21c2464290d\"},{\"content\":{\"connectorIds\":[\"Out1\"],\"side\":\"BOTTOM\"},\"type\":\"ConnectorPlacement.EquallySpacedRectSide\",\"uuid\":\"976aabfd-697c-47ce-8be7-acff7370fc8c\"}]},\"type\":\"ConnectorPlacement.EquallySpacedConnector\",\"uuid\":\"03aa7740-1fdb-47bb-9a21-844669f6bcda\"}],\"packageUris\":[\"http://schema.mathworks.com/mf0/Connector/R2020b\"],\"version\":\"1.0\"}"
      mask Display: disp('vi abc')
  Mjerenje struje4 : Subsystem  Commented=on
      settings: PortSchema="{\"entries\":[{\"content\":{\"sides\":[{\"content\":{\"connectorIds\":[\"LConn1\"]},\"type\":\"ConnectorPlacement.EquallySpacedRectSide\",\"uuid\":\"6fa7c16c-6de5-49c8-bc22-739ef8014510\"},{\"content\":{\"connectorIds\":[\"RConn1\"],\"side\":\"RIGHT\"},\"type\":\"ConnectorPlacement.EquallySpacedRectSide\",\"uuid\":\"6cbb3fe1-95dc-4f03-932b-ab8cb637a208\"},{\"content\":{\"connectorIds\":[\"In1\"],\"side\":\"TOP\"},\"type\":\"ConnectorPlacement.EquallySpacedRectSide\",\"uuid\":\"35a7ae71-901f-47d3-ac0b-d21c2464290d\"},{\"content\":{\"connectorIds\":[\"Out1\"],\"side\":\"BOTTOM\"},\"type\":\"ConnectorPlacement.EquallySpacedRectSide\",\"uuid\":\"976aabfd-697c-47ce-8be7-acff7370fc8c\"}]},\"type\":\"ConnectorPlacement.EquallySpacedConnector\",\"uuid\":\"03aa7740-1fdb-47bb-9a21-844669f6bcda\"}],\"packageUris\":[\"http://schema.mathworks.com/mf0/Connector/R2020b\"],\"version\":\"1.0\"}"
      mask Display: disp('vi abc')
  Mjerenje struje5 : Subsystem
      settings: PortSchema="{\"entries\":[{\"content\":{\"sides\":[{\"content\":{\"connectorIds\":[\"LConn1\"]},\"type\":\"ConnectorPlacement.EquallySpacedRectSide\",\"uuid\":\"6fa7c16c-6de5-49c8-bc22-739ef8014510\"},{\"content\":{\"connectorIds\":[\"RConn1\"],\"side\":\"RIGHT\"},\"type\":\"ConnectorPlacement.EquallySpacedRectSide\",\"uuid\":\"6cbb3fe1-95dc-4f03-932b-ab8cb637a208\"},{\"content\":{\"connectorIds\":[\"In1\"],\"side\":\"TOP\"},\"type\":\"ConnectorPlacement.EquallySpacedRectSide\",\"uuid\":\"35a7ae71-901f-47d3-ac0b-d21c2464290d\"},{\"content\":{\"connectorIds\":[\"Out1\"],\"side\":\"BOTTOM\"},\"type\":\"ConnectorPlacement.EquallySpacedRectSide\",\"uuid\":\"976aabfd-697c-47ce-8be7-acff7370fc8c\"}]},\"type\":\"ConnectorPlacement.EquallySpacedConnector\",\"uuid\":\"03aa7740-1fdb-47bb-9a21-844669f6bcda\"}],\"packageUris\":[\"http://schema.mathworks.com/mf0/Connector/R2020b\"],\"version\":\"1.0\"}"
      mask Display: disp('vi abc')
  Mjerenje struje6 : Subsystem  Commented=on
      settings: PortSchema="{\"entries\":[{\"content\":{\"sides\":[{\"content\":{\"connectorIds\":[\"LConn1\"]},\"type\":\"ConnectorPlacement.EquallySpacedRectSide\",\"uuid\":\"6fa7c16c-6de5-49c8-bc22-739ef8014510\"},{\"content\":{\"connectorIds\":[\"RConn1\"],\"side\":\"RIGHT\"},\"type\":\"ConnectorPlacement.EquallySpacedRectSide\",\"uuid\":\"6cbb3fe1-95dc-4f03-932b-ab8cb637a208\"},{\"content\":{\"connectorIds\":[\"In1\"],\"side\":\"TOP\"},\"type\":\"ConnectorPlacement.EquallySpacedRectSide\",\"uuid\":\"35a7ae71-901f-47d3-ac0b-d21c2464290d\"},{\"content\":{\"connectorIds\":[\"Out1\"],\"side\":\"BOTTOM\"},\"type\":\"ConnectorPlacement.EquallySpacedRectSide\",\"uuid\":\"976aabfd-697c-47ce-8be7-acff7370fc8c\"}]},\"type\":\"ConnectorPlacement.EquallySpacedConnector\",\"uuid\":\"03aa7740-1fdb-47bb-9a21-844669f6bcda\"}],\"packageUris\":[\"http://schema.mathworks.com/mf0/Connector/R2020b\"],\"version\":\"1.0\"}"
      mask Display: disp('vi abc')
  PMSM{1,3..4,7} (4 alike) : ee_lib/Electromechanical/Permanent Magnet/PMSM  port_option=ee.enum.threePhasePort.composite  winding_type=ee.enum.statorconnection.wye  machine_param=ee.enum.pmsm.parameterization.constant  nPolePairs=pp  pmflux_param=ee.enum.pmflux.fluxlinkage  pm_flux_linkage=Psir Wb  torque_constant=0.18 N*m/A  back_emf_constant=0.18 V*s/rad  stator_param=ee.enum.statorparam.LdLqL0  Ld=Ls H  Lq=Ls H  idVec=[-200, 0, 200] A  iqVec=[-200, 0, 200] A  LdMatrix=0.0002 * ones(3, 3) H  LqMatrix=0.0002 * ones(3, 3) H  PmMatrix=0.1 * ones(3, 3) Wb  ktMatrix=0.18 * ones(3, 3) N*m/A  keMatrix=0.18 * ones(3, 3) V*s/rad  L0=(Ld+Lq)/2 H  Ls=0.0002 H  Lm=-0.00002 H  Ms=0.00002 H  Rs=Rs Ohm  zero_sequence=ee.enum.park.zerosequence.exclude  axes_param=ee.enum.rotorangle.daxis  loss_param=ee.enum.ironloss.none  losses_oc=[0, 0, 0] W  losses_sc=[0, 0, 0] W  f_losses=60 Hz  Isc_losses=95 A  J=J kg*m^2  lam=D N*m*s/rad  i_d_specify=off  i_d_priority=None  i_d=0 A  i_d_nominal_specify=off  i_d_nominal_value=1  i_d_nominal_unit=A  i_q_specify=off  i_q_priority=High  i_q=7.1 A  i_q_nominal_specify=on  i_q_nominal_value=7.1  i_q_nominal_unit=A  torque_specify=off  torque_priority=None  torque=0 N*m  torque_nominal_specify=on  torque_nominal_value=Mn  torque_nominal_unit=N*m  angular_velocity_specify=off  angular_velocity_priority=High  angular_velocity=0 rpm  angular_velocity_nominal_specify=on  angular_velocity_nominal_value=6000  angular_velocity_nominal_unit=rpm  angular_position_specify=off  angular_position_priority=High  angular_position=0 deg  angular_position_nominal_specify=off  angular_position_nominal_value=1  angular_position_nominal_unit=deg  alpha=3.93e-3 1/K  alpha_flux=-0.001 1/K  Tmeas=298.15 K  stator_thermal_mass=100 J/K  rotor_thermal_mass=200 J/K  Rm_percent_rotor=90  Rd_percent_rotor=30  temperatureA_specify=off  temperatureA_priority=High  temperatureA=25 degC  temperatureA_nominal_specify=off  temperatureA_nominal_value=1  temperatureA_nominal_unit=degC  temperatureB_specify=off  temperatureB_priority=High  temperatureB=25 degC  temperatureB_nominal_specify=off  temperatureB_nominal_value=1  temperatureB_nominal_unit=degC  temperatureC_specify=off  temperatureC_priority=High  temperatureC=25 degC  temperatureC_nominal_specify=off  temperatureC_nominal_value=1  temperatureC_nominal_unit=degC  temperatureR_specify=off  temperatureR_priority=High  temperatureR=25 degC  temperatureR_nominal_specify=off  temperatureR_nominal_value=1  temperatureR_nominal_unit=degC
  PMSM2 : ee_lib/Electromechanical/Permanent Magnet/PMSM  Commented=on  port_option=ee.enum.threePhasePort.composite  winding_type=ee.enum.statorconnection.wye  machine_param=ee.enum.pmsm.parameterization.constant  nPolePairs=pp  pmflux_param=ee.enum.pmflux.fluxlinkage  pm_flux_linkage=Psir Wb  torque_constant=0.18 N*m/A  back_emf_constant=0.18 V*s/rad  stator_param=ee.enum.statorparam.LdLqL0  Ld=Ls H  Lq=Ls H  idVec=[-200, 0, 200] A  iqVec=[-200, 0, 200] A  LdMatrix=0.0002 * ones(3, 3) H  LqMatrix=0.0002 * ones(3, 3) H  PmMatrix=0.1 * ones(3, 3) Wb  ktMatrix=0.18 * ones(3, 3) N*m/A  keMatrix=0.18 * ones(3, 3) V*s/rad  L0=(Ld+Lq)/2 H  Ls=0.0002 H  Lm=-0.00002 H  Ms=0.00002 H  Rs=Rs Ohm  zero_sequence=ee.enum.park.zerosequence.exclude  axes_param=ee.enum.rotorangle.daxis  loss_param=ee.enum.ironloss.none  losses_oc=[0, 0, 0] W  losses_sc=[0, 0, 0] W  f_losses=60 Hz  Isc_losses=95 A  J=J kg*m^2  lam=D N*m*s/rad  i_d_specify=off  i_d_priority=None  i_d=0 A  i_d_nominal_specify=off  i_d_nominal_value=1  i_d_nominal_unit=A  i_q_specify=off  i_q_priority=High  i_q=7.1 A  i_q_nominal_specify=on  i_q_nominal_value=7.1  i_q_nominal_unit=A  torque_specify=off  torque_priority=None  torque=0 N*m  torque_nominal_specify=on  torque_nominal_value=Mn  torque_nominal_unit=N*m  angular_velocity_specify=off  angular_velocity_priority=High  angular_velocity=0 rpm  angular_velocity_nominal_specify=on  angular_velocity_nominal_value=6000  angular_velocity_nominal_unit=rpm  angular_position_specify=off  angular_position_priority=High  angular_position=0 deg  angular_position_nominal_specify=off  angular_position_nominal_value=1  angular_position_nominal_unit=deg  alpha=3.93e-3 1/K  alpha_flux=-0.001 1/K  Tmeas=298.15 K  stator_thermal_mass=100 J/K  rotor_thermal_mass=200 J/K  Rm_percent_rotor=90  Rd_percent_rotor=30  temperatureA_specify=off  temperatureA_priority=High  temperatureA=25 degC  temperatureA_nominal_specify=off  temperatureA_nominal_value=1  temperatureA_nominal_unit=degC  temperatureB_specify=off  temperatureB_priority=High  temperatureB=25 degC  temperatureB_nominal_specify=off  temperatureB_nominal_value=1  temperatureB_nominal_unit=degC  temperatureC_specify=off  temperatureC_priority=High  temperatureC=25 degC  temperatureC_nominal_specify=off  temperatureC_nominal_value=1  temperatureC_nominal_unit=degC  temperatureR_specify=off  temperatureR_priority=High  temperatureR=25 degC  temperatureR_nominal_specify=off  temperatureR_nominal_value=1  temperatureR_nominal_unit=degC
  PMSM5 : ee_lib/Electromechanical/Permanent Magnet/PMSM  Commented=on  port_option=ee.enum.threePhasePort.composite  winding_type=ee.enum.statorconnection.wye  machine_param=ee.enum.pmsm.parameterization.constant  nPolePairs=pp  pmflux_param=ee.enum.pmflux.fluxlinkage  pm_flux_linkage=Psir Wb  torque_constant=0.18 N*m/A  back_emf_constant=0.18 V*s/rad  stator_param=ee.enum.statorparam.LdLqL0  Ld=Ls H  Lq=Ls H  idVec=[-200, 0, 200] A  iqVec=[-200, 0, 200] A  LdMatrix=0.0002 * ones(3, 3) H  LqMatrix=0.0002 * ones(3, 3) H  PmMatrix=0.1 * ones(3, 3) Wb  ktMatrix=0.18 * ones(3, 3) N*m/A  keMatrix=0.18 * ones(3, 3) V*s/rad  L0=(Ld+Lq)/2 H  Ls=0.0002 H  Lm=-0.00002 H  Ms=0.00002 H  Rs=Rs Ohm  zero_sequence=ee.enum.park.zerosequence.exclude  axes_param=ee.enum.rotorangle.daxis  loss_param=ee.enum.ironloss.none  losses_oc=[0, 0, 0] W  losses_sc=[0, 0, 0] W  f_losses=60 Hz  Isc_losses=95 A  J=J kg*m^2  lam=D N*m*s/rad  i_d_specify=off  i_d_priority=None  i_d=0 A  i_d_nominal_specify=off  i_d_nominal_value=1  i_d_nominal_unit=A  i_q_specify=off  i_q_priority=High  i_q=7.1 A  i_q_nominal_specify=on  i_q_nominal_value=7.1  i_q_nominal_unit=A  torque_specify=off  torque_priority=None  torque=0 N*m  torque_nominal_specify=on  torque_nominal_value=Mn  torque_nominal_unit=N*m  angular_velocity_specify=off  angular_velocity_priority=High  angular_velocity=0 rpm  angular_velocity_nominal_specify=on  angular_velocity_nominal_value=6000  angular_velocity_nominal_unit=rpm  angular_position_specify=off  angular_position_priority=High  angular_position=0 deg  angular_position_nominal_specify=off  angular_position_nominal_value=1  angular_position_nominal_unit=deg  alpha=3.93e-3 1/K  alpha_flux=-0.001 1/K  Tmeas=298.15 K  stator_thermal_mass=100 J/K  rotor_thermal_mass=200 J/K  Rm_percent_rotor=90  Rd_percent_rotor=30  temperatureA_specify=off  temperatureA_priority=High  temperatureA=25 degC  temperatureA_nominal_specify=off  temperatureA_nominal_value=1  temperatureA_nominal_unit=degC  temperatureB_specify=off  temperatureB_priority=High  temperatureB=25 degC  temperatureB_nominal_specify=off  temperatureB_nominal_value=1  temperatureB_nominal_unit=degC  temperatureC_specify=off  temperatureC_priority=High  temperatureC=25 degC  temperatureC_nominal_specify=off  temperatureC_nominal_value=1  temperatureC_nominal_unit=degC  temperatureR_specify=off  temperatureR_priority=High  temperatureR=25 degC  temperatureR_nominal_specify=off  temperatureR_nominal_value=1  temperatureR_nominal_unit=degC
  PWM inverter1 : Subsystem
  PWM inverter2 : Subsystem  Commented=on
  PWM inverter3 : Subsystem
  PWM inverter4 : Subsystem
  PWM inverter5 : Subsystem  Commented=on
  PWM inverter7 : Subsystem
  Rate Transition{1..7,11} (8 alike) : RateTransition  OutPortSampleTime=Ts_current
  Rate Transition{8..10,12} (4 alike) : RateTransition  Commented=on  OutPortSampleTime=Ts_current
  Scope{,1,3,5..6,8..9,11,13..16,18,20..21,23,25..28} (20 alike) : Scope  NumInputPorts=2
      Scope settings: ActiveDisplayYMinimum=-375.02762302228257  ActiveDisplayYMaximum=3375.2486072005436
      Scope1 settings: ActiveDisplayYMinimum=-0.52724313500265274  ActiveDisplayYMaximum=4.7451882150238758  DataLoggingVariableName=ScopeData6
      Scope11 settings: ActiveDisplayYMinimum=501.43236215765944  ActiveDisplayYMaximum=859.41668463074711  DataLoggingVariableName=ScopeData15
      Scope13 settings: ActiveDisplayYMinimum=-274.10667777849955  ActiveDisplayYMaximum=2466.9601000064963  DataLoggingVariableName=ScopeData17
      Scope14 settings: ActiveDisplayYMinimum=-0.51413414630907539  ActiveDisplayYMaximum=7.2788214815531873  DataLoggingVariableName=ScopeData18
      Scope15 settings: ActiveDisplayYMinimum=-375.02762302228257  ActiveDisplayYMaximum=3375.2486072005436  DataLoggingVariableName=ScopeData21
      Scope16 settings: ActiveDisplayYMinimum=-0.52724313500265274  ActiveDisplayYMaximum=4.7451882150238758  DataLoggingVariableName=ScopeData22
      Scope18 settings: ActiveDisplayYMinimum=501.43236215765944  ActiveDisplayYMaximum=859.41668463074711  DataLoggingVariableName=ScopeData24
      Scope20 settings: ActiveDisplayYMinimum=-274.10667777849955  ActiveDisplayYMaximum=2466.9601000064963  DataLoggingVariableName=ScopeData26
      Scope21 settings: ActiveDisplayYMinimum=-0.51413414630907539  ActiveDisplayYMaximum=7.2788214815531873  DataLoggingVariableName=ScopeData27
      Scope23 settings: ActiveDisplayYMinimum=501.43236215765944  ActiveDisplayYMaximum=859.41668463074711  DataLoggingVariableName=ScopeData29
      Scope25 settings: ActiveDisplayYMinimum=-274.10667777849955  ActiveDisplayYMaximum=2466.9601000064963  DataLoggingVariableName=ScopeData31
      Scope26 settings: ActiveDisplayYMinimum=-0.51413414630907539  ActiveDisplayYMaximum=7.2788214815531873  DataLoggingVariableName=ScopeData32
      Scope27 settings: ActiveDisplayYMinimum=-375.02762302228257  ActiveDisplayYMaximum=3375.2486072005436  DataLoggingVariableName=ScopeData33
      Scope28 settings: ActiveDisplayYMinimum=-0.5293107373148902  ActiveDisplayYMaximum=4.7637966358340131  DataLoggingVariableName=ScopeData34
      Scope3 settings: ActiveDisplayYMinimum=501.43236215765944  ActiveDisplayYMaximum=859.41668463074711  DataLoggingVariableName=ScopeData8
      Scope5 settings: ActiveDisplayYMinimum=-274.10667777849955  ActiveDisplayYMaximum=2466.9601000064963  DataLoggingVariableName=ScopeData11
      Scope6 settings: ActiveDisplayYMinimum=-0.51413414630907539  ActiveDisplayYMaximum=7.2788214815531873  DataLoggingVariableName=ScopeData12
      Scope8 settings: ActiveDisplayYMinimum=-375.02762302228257  ActiveDisplayYMaximum=3375.2486072005436  DataLoggingVariableName=ScopeData19
      Scope9 settings: ActiveDisplayYMinimum=-0.5293107373148902  ActiveDisplayYMaximum=4.7637966358340131  DataLoggingVariableName=ScopeData20
  Scope{2,4,10,12,17,19,22,24} (8 alike) : Scope
      Scope10 settings: ActiveDisplayYMinimum=-5281.0613442070317  ActiveDisplayYMaximum=3730.2587788855749  DataLoggingVariableName=ScopeData14
      Scope12 settings: ActiveDisplayYMinimum=-66.335912940720434  ActiveDisplayYMaximum=63.17125095285094  DataLoggingVariableName=ScopeData16
      Scope17 settings: ActiveDisplayYMinimum=-5281.0613442070317  ActiveDisplayYMaximum=3730.2587788855749  DataLoggingVariableName=ScopeData23
      Scope19 settings: ActiveDisplayYMinimum=-66.335912940720434  ActiveDisplayYMaximum=63.17125095285094  DataLoggingVariableName=ScopeData25
      Scope2 settings: ActiveDisplayYMinimum=-5281.0613442070317  ActiveDisplayYMaximum=3730.2587788855749  DataLoggingVariableName=ScopeData7
      Scope22 settings: ActiveDisplayYMinimum=-5281.0613442070317  ActiveDisplayYMaximum=3730.2587788855749  DataLoggingVariableName=ScopeData28
      Scope24 settings: ActiveDisplayYMinimum=-66.335912940720434  ActiveDisplayYMaximum=63.17125095285094  DataLoggingVariableName=ScopeData30
      Scope4 settings: ActiveDisplayYMinimum=-66.335912940720434  ActiveDisplayYMaximum=63.17125095285094  DataLoggingVariableName=ScopeData9
  Scope{29..30,32,34..37,39,41..42} (10 alike) : Scope  Commented=on  NumInputPorts=2
      Scope29 settings: ActiveDisplayYMinimum=-375.02762302228257  ActiveDisplayYMaximum=3375.2486072005436  DataLoggingVariableName=ScopeData35
      Scope30 settings: ActiveDisplayYMinimum=-0.04083992735226416  ActiveDisplayYMaximum=1.0566345682915843  DataLoggingVariableName=ScopeData36
      Scope32 settings: ActiveDisplayYMinimum=-213.18216528333605  ActiveDisplayYMaximum=457.21724609252726  DataLoggingVariableName=ScopeData38
      Scope34 settings: ActiveDisplayYMinimum=-274.10667777849955  ActiveDisplayYMaximum=2466.9601000064963  DataLoggingVariableName=ScopeData40
      Scope35 settings: ActiveDisplayYMinimum=-0.51413414630907539  ActiveDisplayYMaximum=7.2788214815531873  DataLoggingVariableName=ScopeData41
      Scope36 settings: ActiveDisplayYMinimum=-375.02762302228257  ActiveDisplayYMaximum=3375.2486072005436  DataLoggingVariableName=ScopeData42
      Scope37 settings: ActiveDisplayYMinimum=-0.04083992735226416  ActiveDisplayYMaximum=1.0566345682915843  DataLoggingVariableName=ScopeData43
      Scope39 settings: ActiveDisplayYMinimum=-213.18216528333605  ActiveDisplayYMaximum=457.21724609252726  DataLoggingVariableName=ScopeData45
      Scope41 settings: ActiveDisplayYMinimum=-274.10667777849955  ActiveDisplayYMaximum=2466.9601000064963  DataLoggingVariableName=ScopeData47
      Scope42 settings: ActiveDisplayYMinimum=-0.51413414630907539  ActiveDisplayYMaximum=7.2788214815531873  DataLoggingVariableName=ScopeData48
  Scope{31,33,38,40} (4 alike) : Scope  Commented=on
      Scope31 settings: ActiveDisplayYMinimum=-5281.0613442070317  ActiveDisplayYMaximum=3730.2587788855749  DataLoggingVariableName=ScopeData37
      Scope33 settings: ActiveDisplayYMinimum=-66.335912940720434  ActiveDisplayYMaximum=63.17125095285094  DataLoggingVariableName=ScopeData39
      Scope38 settings: ActiveDisplayYMinimum=-5281.0613442070317  ActiveDisplayYMaximum=3730.2587788855749  DataLoggingVariableName=ScopeData44
      Scope40 settings: ActiveDisplayYMinimum=-66.335912940720434  ActiveDisplayYMaximum=63.17125095285094  DataLoggingVariableName=ScopeData46
  Scope43 : Scope  NumInputPorts=5
      settings: ActiveDisplayYMinimum=-0.12499999999999997  ActiveDisplayYMaximum=1.125  DataLoggingVariableName=ScopeData2
  Scope7 : Scope  NumInputPorts=5
      settings: ActiveDisplayYMinimum=1914.077823494009  ActiveDisplayYMaximum=2070.5085585415382  DataLoggingVariableName=ScopeData13
  Simulink-PS Converter{,1..7} (8 alike) : nesl_utility/Simulink-PS Converter  PhysicalDomain=network_engine_domain  SubClassName=ps_input  LeftPortType=input  RightPortType=output  PseudoPeriodic=off  Frequencies=[]  NoiseDistribution=none  NoiseParameters=[]  Unit=1  AffineConversion=off  FilteringAndDerivatives=provide  SimscapeFilterOrder=1  InputFilterTimeConstant=0.001  UdotUserProvided=0
  Simulink-PS Converter{8..11} (4 alike) : nesl_utility/Simulink-PS Converter  Commented=on  PhysicalDomain=network_engine_domain  SubClassName=ps_input  LeftPortType=input  RightPortType=output  PseudoPeriodic=off  Frequencies=[]  NoiseDistribution=none  NoiseParameters=[]  Unit=1  AffineConversion=off  FilteringAndDerivatives=provide  SimscapeFilterOrder=1  InputFilterTimeConstant=0.001  UdotUserProvided=0
  Solver Configuration{1..3,6} (4 alike) : nesl_utility/Solver Configuration  PhysicalDomain=network_engine_domain  SubClassName=solver  LeftPortType=input  RightPortType=generic  Tones=[]  Harmonics=[]  SimulateNoise=off  Profile=off  UseLocalSampling=off  EnableSwitchedLinearOptims=on  FrequencyDomain=off  UseCCode=off  RelTol=0.001  AbsTol=0.001  MinStep=1e-09  ToWorkspace=off  RevertToSquareIcSolve=off  NumHomotopyIterations=100  PhasorMode=off  PhasorModeNumHarmonics=1  ConsistencySolver=NEWTON_XTOL_AFTER_FTOL  CanonicalOrdering=UNORDERED  OptimizeIntermediates=UNOPTIMIZED  IndexReductionMethod=DerivativeReplacement  DoDC=off  ResidualTolerance=1e-09  ConsistencyTolSource=GLOBAL  ConsistencyAbsTol=0.001  ConsistencyRelTol=0.001  ConsistencyTolFactor=0.001  UseLocalSolver=off  LocalSolverChoice=NE_BACKWARD_EULER_ADVANCER  ResolveIndetEquations=on  FunctionEvalNumThread=1  LocalSolverSampleTime=0.001  DoFixedCost=off  MaxNonlinIter=3  MaxModeIter=2  ComputeImpulses=off  ImpulseIterations=2  LinearAlgebra=auto  LinearAlgebraNumThread=0  EquationFormulation=NE_TIME_EF  DelaysMemoryBudget=1024  AutomaticFiltering=on  FilteringTimeConstant=0.001  PartitionStorageMethod=AS_NEEDED  PartitionMemoryBudget=1024  PartitionMethod=ROBUST  MultibodyUseLocalSolver=off  MultibodyLocalSolverChoice=ODE1  MultibodyLocalSolverSampleTime=0.001
  Solver Configuration4 : nesl_utility/Solver Configuration  Commented=on  PhysicalDomain=network_engine_domain  SubClassName=solver  LeftPortType=input  RightPortType=generic  Tones=[]  Harmonics=[]  SimulateNoise=off  Profile=off  UseLocalSampling=off  EnableSwitchedLinearOptims=on  FrequencyDomain=off  UseCCode=off  RelTol=0.001  AbsTol=0.001  MinStep=1e-09  ToWorkspace=off  RevertToSquareIcSolve=off  NumHomotopyIterations=100  PhasorMode=off  PhasorModeNumHarmonics=1  ConsistencySolver=NEWTON_XTOL_AFTER_FTOL  CanonicalOrdering=UNORDERED  OptimizeIntermediates=UNOPTIMIZED  IndexReductionMethod=DerivativeReplacement  DoDC=off  ResidualTolerance=1e-09  ConsistencyTolSource=GLOBAL  ConsistencyAbsTol=0.001  ConsistencyRelTol=0.001  ConsistencyTolFactor=0.001  UseLocalSolver=off  LocalSolverChoice=NE_BACKWARD_EULER_ADVANCER  ResolveIndetEquations=on  FunctionEvalNumThread=1  LocalSolverSampleTime=0.001  DoFixedCost=off  MaxNonlinIter=3  MaxModeIter=2  ComputeImpulses=off  ImpulseIterations=2  LinearAlgebra=auto  LinearAlgebraNumThread=0  EquationFormulation=NE_TIME_EF  DelaysMemoryBudget=1024  AutomaticFiltering=on  FilteringTimeConstant=0.001  PartitionStorageMethod=AS_NEEDED  PartitionMemoryBudget=1024  PartitionMethod=ROBUST  MultibodyUseLocalSolver=off  MultibodyLocalSolverChoice=ODE1  MultibodyLocalSolverSampleTime=0.001
  Solver Configuration5 : nesl_utility/Solver Configuration  Commented=on  PhysicalDomain=network_engine_domain  SubClassName=solver  LeftPortType=input  RightPortType=generic  Tones=[]  Harmonics=[]  SimulateNoise=off  Profile=off  UseLocalSampling=off  EnableSwitchedLinearOptims=on  FrequencyDomain=off  UseCCode=off  RelTol=0.001  AbsTol=0.001  MinStep=1e-09  ToWorkspace=off  RevertToSquareIcSolve=off  NumHomotopyIterations=100  PhasorMode=off  PhasorModeNumHarmonics=1  ConsistencySolver=NEWTON_XTOL_AFTER_FTOL  CanonicalOrdering=UNORDERED  OptimizeIntermediates=UNOPTIMIZED  IndexReductionMethod=DerivativeReplacement  DoDC=off  ResidualTolerance=1e-09  ConsistencyTolSource=GLOBAL  ConsistencyAbsTol=0.001  ConsistencyRelTol=0.001  ConsistencyTolFactor=0.001  UseLocalSolver=off  LocalSolverChoice=NE_BACKWARD_EULER_ADVANCER  ResolveIndetEquations=on  FunctionEvalNumThread=1  LocalSolverSampleTime=0.001  DoFixedCost=off  MaxNonlinIter=3  MaxModeIter=2  ComputeImpulses=off  ImpulseIterations=2  LinearAlgebra=auto  LinearAlgebraNumThread=0  EquationFormulation=NE_TIME_EF  DelaysMemoryBudget=1024  AutomaticFiltering=on  FilteringTimeConstant=0.001  PartitionStorageMethod=AS_NEEDED  PartitionMemoryBudget=1024  PartitionMethod=ROBUST  MultibodyUseLocalSolver=off  MultibodyLocalSolverChoice=ODE1  MultibodyLocalSolverSampleTime=0.001
  Step : Step  Time=0.5  FinalValue=-1200  SampleTime=0
  Step{1..4} (4 alike) : Step  Time=1.5  FinalValue=-Mn/2  SampleTime=0
  Step10 : Step  Commented=on  Time=0.1  FinalValue=1000  SampleTime=0
  Step11 : Step  Time=0  SampleTime=0
  Step5 : Step  Commented=on  Time=1.5  FinalValue=-Mn/2  SampleTime=0
  Step6 : Step  Commented=on  Time=0.1  SampleTime=0
  Step7 : Step  Commented=on  Time=0.1  FinalValue=1000  SampleTime=0
  Step8 : Step  Commented=on  Time=1.5  FinalValue=-Mn/2  SampleTime=0
  Step9 : Step  Commented=on  Time=0.1  SampleTime=0
  Sum : Sum  Inputs=|++
  Terminator{1..6,12..13} (8 alike) : Terminator
  Terminator{7..10} (4 alike) : Terminator  Commented=on
  To Workspace : ToWorkspace  Commented=on  VariableName=current_emulation_backeuler  SaveFormat=Timeseries  SampleTime=-1
  To Workspace1 : ToWorkspace  Commented=on  VariableName=current_emulation_tustin  SaveFormat=Timeseries  SampleTime=-1
  To Workspace2 : ToWorkspace  Commented=on  VariableName=current_direct_backeuler  SaveFormat=Timeseries  SampleTime=-1
  To Workspace3 : ToWorkspace  Commented=on  VariableName=current_direct_tustin  SaveFormat=Timeseries  SampleTime=-1
  To Workspace4 : ToWorkspace  VariableName=n_emulation_backeuler  SaveFormat=Timeseries  SampleTime=-1
  To Workspace5 : ToWorkspace  VariableName=n_emulation_tustin  SaveFormat=Timeseries  SampleTime=-1
  To Workspace6 : ToWorkspace  VariableName=n_direct_backeuler  SaveFormat=Timeseries  SampleTime=-1
  To Workspace7 : ToWorkspace  VariableName=n_direct_tustin  SaveFormat=Timeseries  SampleTime=-1
  To Workspace8 : ToWorkspace  Commented=on  VariableName=current_ref  SaveFormat=Timeseries  SampleTime=-1
  To Workspace9 : ToWorkspace  VariableName=n_ref  SaveFormat=Timeseries  SampleTime=-1
  Unit Delay{,1..24} (25 alike) : UnitDelay  SampleTime=Ts_current
  Unit Delay{25..38} (14 alike) : UnitDelay  Commented=on  SampleTime=Ts_current
  n_ref : Step  Time=0  FinalValue=2000  SampleTime=0
  wires:
  Diskretni regulatori struje5/2(uq_ref) -> PWM inverter7/2(uq_ref)
  Demux7/2 -> [i_disc_emu_tustin], Scope1/2, Diskretni regulatori struje5/4(iq_mj)
  Rate Transition11/1 -> Demux7/1
  PWM inverter7/1(u_abc*) -> Simulink-PS Converter6/1
  Demux7/1 -> Diskretni regulatori struje5/3(id_mj)
  Mjerenje kuta i brzine6/2(theta_e) -> Scope6/2, Encoder/1(angle)
  Diskretni regulatori struje5/1(ud_ref) -> PWM inverter7/1(ud_ref)
  Demux7/3 -> Terminator12/1
  Mjerenje momenta6/1(Output) -> Terminator13/1
  Mjerenje struje5/1(Output) -> Rate Transition11/1
  Mjerenje kuta i brzine6/1(we) -> Rate Transition5/1
  [i_ref] -> Scope43/1  "i_ref"
  Rate Transition5/1 -> Scope2/1, [we_tustin_emulation], Scope5/2, Diskretni regulatori struje5/5(we)
  Unit Delay/1 -> Encoder/2(angle_prev)
  Encoder/3(q_angle) -> Unit Delay/1
  Constant/1 -> Diskretni regulatori struje5/1(id_ref)
  Encoder/1(theta_e) -> Scope6/1, [theta_e_tustin_emulation], Scope/1
  Encoder/2(omega_e) -> Low-Pass Filter Speed/1(x), Scope/2
  Low-Pass Filter Speed/2(y_prev_out) -> Unit Delay1/1
  Unit Delay1/1 -> Low-Pass Filter Speed/2(y_prev)
  Low-Pass Filter Speed/1(y) -> [w_filtered_tustin_emulation], Scope5/1
  Low-Pass Filter Speed/3(x_prev_out) -> Unit Delay2/1
  Unit Delay2/1 -> Low-Pass Filter Speed/3(x_prev)
  Diskretni regulator brzine5/1(iq_ref) -> Low-Pass Filter Current/1(x), Scope4/1
  Manual Switch7/1 -> Scope1/1, Diskretni regulatori struje5/2(iq_ref)
  Low-Pass Filter Current/1(y) -> Manual Switch7/2
  Low-Pass Filter Current/2(y_prev_out) -> Unit Delay4/1
  Unit Delay4/1 -> Low-Pass Filter Current/2(y_prev)
  Low-Pass Filter Current/3(x_prev_out) -> Unit Delay3/1
  Unit Delay3/1 -> Low-Pass Filter Current/3(x_prev)
  Sum/1 -> [n_ref], Gain1/1
  n_ref/1 -> Sum/1
  Gain1/1 -> Low-Pass Filter Speed Ref/1(x)
  Low-Pass Filter Speed Ref/1(y) -> Scope3/1, Diskretni regulator brzine5/1(w_ref)
  Low-Pass Filter Speed Ref/2(y_prev_out) -> Unit Delay5/1
  Unit Delay5/1 -> Low-Pass Filter Speed Ref/2(y_prev)
  Low-Pass Filter Speed Ref/3(x_prev_out) -> Unit Delay6/1
  Unit Delay6/1 -> Low-Pass Filter Speed Ref/3(x_prev)
  Step1/1 -> Simulink-PS Converter/1
  Manual Switch/1 -> Diskretni regulator brzine5/2(w_mj), Gain2/1, Scope3/2
  [w_filtered_tustin_emulation] -> Manual Switch/1
  [we_tustin_emulation] -> Manual Switch/2
  [theta_e_tustin_emulation] -> Mjerenje struje5/1(Input)
  [theta_e_tustin_emulation] -> PWM inverter7/3(theta_e_mj)
  Constant2/1 -> Low-Pass Filter Speed/4(fc)
  Constant3/1 -> Low-Pass Filter Speed/5(TS)
  Constant4/1 -> Encoder/3(N)
  Constant5/1 -> Encoder/4(dt)
  Constant6/1 -> Encoder/5(pole_pairs)
  Constant7/1 -> Low-Pass Filter Current/4(fc)
  Constant8/1 -> Low-Pass Filter Current/5(TS)
  Constant9/1 -> Low-Pass Filter Speed Ref/4(fc)
  Constant11/1 -> Low-Pass Filter Speed Ref/5(TS)
  Gain2/1 -> [n_tustin_emulation]
  [n_ref] -> Scope7/1
  Constant15/1 -> Encoder1/4(dt)
  Constant16/1 -> Encoder1/5(pole_pairs)
  Constant14/1 -> Encoder1/3(N)
  [theta_e_tustin_direct] -> Mjerenje struje2/1(Input)
  Constant18/1 -> Low-Pass Filter Current1/5(TS)
  [we_tustin_direct] -> Manual Switch1/2
  Constant17/1 -> Low-Pass Filter Current1/4(fc)
  Constant12/1 -> Low-Pass Filter Speed1/4(fc)
  Gain4/1 -> [n_tustin_direct]
  Unit Delay13/1 -> Low-Pass Filter Speed Ref1/3(x_prev)
  Gain3/1 -> Low-Pass Filter Speed Ref1/1(x)
  Step3/1 -> Simulink-PS Converter3/1
  Constant13/1 -> Low-Pass Filter Speed1/5(TS)
  Low-Pass Filter Current1/2(y_prev_out) -> Unit Delay11/1
  Low-Pass Filter Speed Ref1/2(y_prev_out) -> Unit Delay12/1
  Manual Switch2/1 -> Scope9/1, Diskretni regulatori struje2/2(iq_ref)
  Low-Pass Filter Speed Ref1/1(y) -> Scope11/1, Diskretni regulator brzine1/1(w_ref)
  Constant19/1 -> Low-Pass Filter Speed Ref1/4(fc)
  Unit Delay12/1 -> Low-Pass Filter Speed Ref1/2(y_prev)
  Unit Delay10/1 -> Low-Pass Filter Current1/3(x_prev)
  Low-Pass Filter Speed Ref1/3(x_prev_out) -> Unit Delay13/1
  Manual Switch1/1 -> Diskretni regulator brzine1/2(w_mj), Gain4/1, Scope11/2
  Constant1/1 -> Diskretni regulatori struje2/1(id_ref)
  Encoder1/1(theta_e) -> Scope14/1, [theta_e_tustin_direct], Scope8/1
  Diskretni regulator brzine1/1(iq_ref) -> Low-Pass Filter Current1/1(x), Scope12/1
  [w_filtered_tustin_direct] -> Manual Switch1/1
  Demux4/1 -> Diskretni regulatori struje2/3(id_mj)
  Rate Transition4/1 -> Scope10/1, [we_tustin_direct], Scope13/2, Diskretni regulatori struje2/5(we)
  Unit Delay9/1 -> Low-Pass Filter Speed1/3(x_prev)
  Unit Delay7/1 -> Encoder1/2(angle_prev)
  PWM inverter4/1(u_abc*) -> Simulink-PS Converter7/1
  Mjerenje momenta3/1(Output) -> Terminator6/1
  Demux4/2 -> [i_direct_tustin], Scope9/2, Diskretni regulatori struje2/4(iq_mj)
  Encoder1/2(omega_e) -> Low-Pass Filter Speed1/1(x), Scope8/2
  Unit Delay11/1 -> Low-Pass Filter Current1/2(y_prev)
  Mjerenje kuta i brzine3/2(theta_e) -> Scope14/2, Encoder1/1(angle)
  Diskretni regulatori struje2/1(ud_ref) -> PWM inverter4/1(ud_ref)
  Low-Pass Filter Speed1/2(y_prev_out) -> Unit Delay8/1
  Low-Pass Filter Speed1/1(y) -> [w_filtered_tustin_direct], Scope13/1
  Demux4/3 -> Terminator5/1
  Rate Transition3/1 -> Demux4/1
  Low-Pass Filter Current1/3(x_prev_out) -> Unit Delay10/1
  Low-Pass Filter Current1/1(y) -> Manual Switch2/2
  [theta_e_tustin_direct] -> PWM inverter4/3(theta_e_mj)
  Diskretni regulatori struje2/2(uq_ref) -> PWM inverter4/2(uq_ref)
  Mjerenje kuta i brzine3/1(we) -> Rate Transition4/1
  Encoder1/3(q_angle) -> Unit Delay7/1
  Unit Delay8/1 -> Low-Pass Filter Speed1/2(y_prev)
  Constant10/1 -> Low-Pass Filter Speed Ref1/5(TS)
  Mjerenje struje2/1(Output) -> Rate Transition3/1
  Low-Pass Filter Speed1/3(x_prev_out) -> Unit Delay9/1
  [n_ref] -> Gain3/1
  Constant25/1 -> Encoder2/4(dt)
  Constant26/1 -> Encoder2/5(pole_pairs)
  Constant24/1 -> Encoder2/3(N)
  [theta_e_backeuler_emulation] -> Mjerenje struje1/1(Input)
  Constant28/1 -> Low-Pass Filter Current2/4(TS)
  [we_backeuler_emulation] -> Manual Switch3/2
  Constant27/1 -> Low-Pass Filter Current2/3(fc)
  Gain6/1 -> [n_backeuler_emulation]
  Gain5/1 -> Low-Pass Filter Speed Ref2/1(x)
  Step4/1 -> Simulink-PS Converter1/1
  Low-Pass Filter Current2/2(y_prev_out) -> Unit Delay18/1
  Low-Pass Filter Speed Ref2/2(y_prev_out) -> Unit Delay19/1
  Manual Switch4/1 -> Scope16/1, Diskretni regulatori struje1/2(iq_ref)
  Low-Pass Filter Speed Ref2/1(y) -> Scope18/1, Diskretni regulator brzine2/1(w_ref)
  Constant29/1 -> Low-Pass Filter Speed Ref2/3(fc)
  Unit Delay19/1 -> Low-Pass Filter Speed Ref2/2(y_prev)
  Manual Switch3/1 -> Diskretni regulator brzine2/2(w_mj), Gain6/1, Scope18/2
  Constant20/1 -> Diskretni regulatori struje1/1(id_ref)
  Encoder2/1(theta_e) -> Scope21/1, [theta_e_backeuler_emulation], Scope15/1
  Diskretni regulator brzine2/1(iq_ref) -> Low-Pass Filter Current2/1(x), Scope19/1
  [w_filtered_backeuler_emulation] -> Manual Switch3/1
  Demux3/1 -> Diskretni regulatori struje1/3(id_mj)
  Rate Transition7/1 -> [we_backeuler_emulation], Scope20/2, Diskretni regulatori struje1/5(we), Scope17/1
  Unit Delay14/1 -> Encoder2/2(angle_prev)
  PWM inverter3/1(u_abc*) -> Simulink-PS Converter5/1
  Mjerenje momenta2/1(Output) -> Terminator4/1
  Demux3/2 -> [i_disc_emu_back], Scope16/2, Diskretni regulatori struje1/4(iq_mj)
  Encoder2/2(omega_e) -> Low-Pass Filter Speed2/1(x), Scope15/2
  Unit Delay18/1 -> Low-Pass Filter Current2/2(y_prev)
  Mjerenje kuta i brzine2/2(theta_e) -> Scope21/2, Encoder2/1(angle)
  Diskretni regulatori struje1/1(ud_ref) -> PWM inverter3/1(ud_ref)
  Low-Pass Filter Speed2/2(y_prev_out) -> Unit Delay15/1
  Low-Pass Filter Speed2/1(y) -> [w_filtered_backeuler_emulation], Scope20/1
  Demux3/3 -> Terminator3/1
  Rate Transition2/1 -> Demux3/1
  Low-Pass Filter Current2/1(y) -> Manual Switch4/2
  [theta_e_backeuler_emulation] -> PWM inverter3/3(theta_e_mj)
  Diskretni regulatori struje1/2(uq_ref) -> PWM inverter3/2(uq_ref)
  Mjerenje kuta i brzine2/1(we) -> Rate Transition7/1
  Encoder2/3(q_angle) -> Unit Delay14/1
  Unit Delay15/1 -> Low-Pass Filter Speed2/2(y_prev)
  Constant21/1 -> Low-Pass Filter Speed Ref2/4(TS)
  Mjerenje struje1/1(Output) -> Rate Transition2/1
  Constant23/1 -> Low-Pass Filter Speed2/4(TS)
  Constant22/1 -> Low-Pass Filter Speed2/3(fc)
  [n_ref] -> Gain5/1
  Mjerenje kuta i brzine1/1(we) -> Rate Transition6/1
  [theta_e_backeuler_direct] -> PWM inverter1/3(theta_e_mj)
  Encoder3/3(q_angle) -> Unit Delay22/1
  Low-Pass Filter Current3/3(x_prev_out) -> Unit Delay16/1
  Low-Pass Filter Speed3/1(y) -> [w_filtered_backeuler_direct], Scope25/1
  Low-Pass Filter Current3/1(y) -> Manual Switch6/2
  Demux1/3 -> Terminator1/1
  Low-Pass Filter Speed3/2(y_prev_out) -> Unit Delay23/1
  Mjerenje kuta i brzine1/2(theta_e) -> Scope26/2, Encoder3/1(angle)
  Unit Delay17/1 -> Low-Pass Filter Current3/2(y_prev)
  Diskretni regulatori struje3/1(ud_ref) -> PWM inverter1/1(ud_ref)
  Demux1/2 -> [i_direct_back], Scope28/2, Diskretni regulatori struje3/4(iq_mj)
  Unit Delay22/1 -> Encoder3/2(angle_prev)
  PWM inverter1/1(u_abc*) -> Simulink-PS Converter4/1
  Encoder3/2(omega_e) -> Low-Pass Filter Speed3/1(x), Scope27/2
  Mjerenje momenta1/1(Output) -> Terminator2/1
  Unit Delay24/1 -> Low-Pass Filter Speed3/3(x_prev)
  Rate Transition1/1 -> Demux1/1
  [w_filtered_backeuler_direct] -> Manual Switch5/1
  Diskretni regulator brzine3/1(iq_ref) -> Low-Pass Filter Current3/1(x), Scope24/1
  Rate Transition6/1 -> Scope22/1, [we_backeuler_direct], Scope25/2, Diskretni regulatori struje3/5(we)
  Unit Delay20/1 -> Low-Pass Filter Speed Ref3/2(y_prev)
  Demux1/1 -> Diskretni regulatori struje3/3(id_mj)
  Low-Pass Filter Speed Ref3/3(x_prev_out) -> Unit Delay21/1
  Constant31/1 -> Low-Pass Filter Speed Ref3/5(TS)
  Mjerenje struje3/1(Output) -> Rate Transition1/1
  Constant30/1 -> Diskretni regulatori struje3/1(id_ref)
  Constant39/1 -> Low-Pass Filter Speed Ref3/4(fc)
  Diskretni regulatori struje3/2(uq_ref) -> PWM inverter1/2(uq_ref)
  Low-Pass Filter Current3/2(y_prev_out) -> Unit Delay17/1
  Low-Pass Filter Speed Ref3/1(y) -> Scope23/1, Diskretni regulator brzine3/1(w_ref)
  Manual Switch6/1 -> Scope28/1, Diskretni regulatori struje3/2(iq_ref)
  Low-Pass Filter Speed3/3(x_prev_out) -> Unit Delay24/1
  Manual Switch5/1 -> Diskretni regulator brzine3/2(w_mj), Gain15/1, Scope23/2
  Low-Pass Filter Speed Ref3/2(y_prev_out) -> Unit Delay20/1
  Gain15/1 -> [n_backeuler_direct]
  Unit Delay16/1 -> Low-Pass Filter Current3/3(x_prev)
  Constant33/1 -> Low-Pass Filter Speed3/5(TS)
  Encoder3/1(theta_e) -> Scope26/1, [theta_e_backeuler_direct], Scope27/1
  Gain7/1 -> Low-Pass Filter Speed Ref3/1(x)
  Step2/1 -> Simulink-PS Converter2/1
  Unit Delay21/1 -> Low-Pass Filter Speed Ref3/3(x_prev)
  Constant32/1 -> Low-Pass Filter Speed3/4(fc)
  Constant37/1 -> Low-Pass Filter Current3/4(fc)
  Constant35/1 -> Encoder3/4(dt)
  [we_backeuler_direct] -> Manual Switch5/2
  Constant36/1 -> Encoder3/5(pole_pairs)
  Constant34/1 -> Encoder3/3(N)
  Constant38/1 -> Low-Pass Filter Current3/5(TS)
  Unit Delay23/1 -> Low-Pass Filter Speed3/2(y_prev)
  [theta_e_backeuler_direct] -> Mjerenje struje3/1(Input)
  [n_ref] -> Gain7/1
  Mjerenje struje4/1(Output) -> Rate Transition8/1
  Encoder4/3(q_angle) -> Unit Delay25/1
  Unit Delay26/1 -> Low-Pass Filter Speed4/2(y_prev)
  Constant41/1 -> Low-Pass Filter Speed Ref4/5(TS)
  Mjerenje kuta i brzine4/1(we) -> Rate Transition9/1
  From32/1 -> PWM inverter2/3(theta_e_mj)
  Rate Transition8/1 -> Demux2/1
  Diskretni regulatori struje4/2(uq_ref) -> PWM inverter2/2(uq_ref)
  Demux2/3 -> Terminator7/1
  Low-Pass Filter Speed4/1(y) -> Scope34/1, Goto18/1
  Low-Pass Filter Speed4/2(y_prev_out) -> Unit Delay26/1
  Mjerenje kuta i brzine4/2(theta_e) -> Scope35/2, Encoder4/1(angle)
  Low-Pass Filter Current4/1(y) -> Manual Switch9/2
  Diskretni regulatori struje4/1(ud_ref) -> PWM inverter2/1(ud_ref)
  Encoder4/2(omega_e) -> Low-Pass Filter Speed4/1(x), Scope29/2
  Mjerenje momenta4/1(Output) -> Terminator8/1
  Unit Delay27/1 -> Low-Pass Filter Current4/2(y_prev)
  From33/1 -> Manual Switch8/1
  Unit Delay25/1 -> Encoder4/2(angle_prev)
  Demux2/1 -> Diskretni regulatori struje4/3(id_mj)
  Diskretni regulator brzine4/1(iq_ref) -> Low-Pass Filter Current4/1(x), Scope33/1
  Constant40/1 -> Diskretni regulatori struje4/1(id_ref)
  Unit Delay28/1 -> Low-Pass Filter Speed Ref4/2(y_prev)
  Low-Pass Filter Speed Ref4/1(y) -> Scope32/1, Diskretni regulator brzine4/1(w_ref)
  Low-Pass Filter Current4/2(y_prev_out) -> Unit Delay27/1
  Gain16/1 -> Low-Pass Filter Speed Ref4/1(x)
  Low-Pass Filter Speed Ref4/2(y_prev_out) -> Unit Delay28/1
  Manual Switch9/1 -> Scope30/1, Diskretni regulatori struje4/2(iq_ref)
  From35/1 -> Manual Switch8/2
  From34/1 -> Mjerenje struje4/1(Input)
  Constant48/1 -> Low-Pass Filter Current4/5(TS)
  Constant47/1 -> Low-Pass Filter Current4/4(fc)
  Constant44/1 -> Encoder4/3(N)
  Constant45/1 -> Encoder4/4(dt)
  Rate Transition9/1 -> Goto19/1, Scope34/2, Diskretni regulatori struje4/5(we), Scope31/1
  PWM inverter2/1(u_abc*) -> Simulink-PS Converter9/1
  Encoder4/1(theta_e) -> Scope35/1, Goto21/1, Scope29/1
  Constant46/1 -> Encoder4/5(pole_pairs)
  Gain17/1 -> Goto20/1
  Step5/1 -> Simulink-PS Converter8/1
  Manual Switch8/1 -> Diskretni regulator brzine4/2(w_mj), Gain17/1, Scope32/2
  Constant49/1 -> Low-Pass Filter Speed Ref4/4(fc)
  Demux2/2 -> Scope30/2, Diskretni regulatori struje4/4(iq_mj)
  Low-Pass Filter Speed4/3(x_prev_out) -> Unit Delay29/1
  Unit Delay29/1 -> Low-Pass Filter Speed4/3(x_prev)
  Constant42/1 -> Low-Pass Filter Speed4/4(fc)
  Constant43/1 -> Low-Pass Filter Speed4/5(TS)
  Low-Pass Filter Speed Ref4/3(x_prev_out) -> Unit Delay30/1
  Unit Delay30/1 -> Low-Pass Filter Speed Ref4/3(x_prev)
  Low-Pass Filter Current4/3(x_prev_out) -> Unit Delay31/1
  Unit Delay31/1 -> Low-Pass Filter Current4/3(x_prev)
  Step6/1 -> Manual Switch9/1
  Step7/1 -> Gain16/1
  Constant53/1 -> Low-Pass Filter Speed5/5(TS)
  From39/1 -> Manual Switch10/1
  Diskretni regulatori struje6/2(uq_ref) -> PWM inverter5/2(uq_ref)
  Gain19/1 -> Goto24/1
  Unit Delay36/1 -> Low-Pass Filter Speed5/3(x_prev)
  From38/1 -> PWM inverter5/3(theta_e_mj)
  From41/1 -> Manual Switch10/2
  Gain18/1 -> Low-Pass Filter Speed Ref5/1(x)
  Manual Switch10/1 -> Diskretni regulator brzine6/2(w_mj), Gain19/1, Scope39/2
  Rate Transition12/1 -> Goto23/1, Scope41/2, Diskretni regulatori struje6/5(we), Scope38/1
  Constant52/1 -> Low-Pass Filter Speed5/4(fc)
  Low-Pass Filter Current5/2(y_prev_out) -> Unit Delay34/1
  Unit Delay35/1 -> Low-Pass Filter Speed Ref5/2(y_prev)
  Constant50/1 -> Diskretni regulatori struje6/1(id_ref)
  Low-Pass Filter Current5/3(x_prev_out) -> Unit Delay38/1
  Low-Pass Filter Current5/1(y) -> Manual Switch11/2
  Step8/1 -> Simulink-PS Converter10/1
  Constant57/1 -> Low-Pass Filter Current5/4(fc)
  Demux5/2 -> Scope37/2, Diskretni regulatori struje6/4(iq_mj)
  Step9/1 -> Manual Switch11/1
  Diskretni regulator brzine6/1(iq_ref) -> Low-Pass Filter Current5/1(x), Scope40/1
  Unit Delay38/1 -> Low-Pass Filter Current5/3(x_prev)
  PWM inverter5/1(u_abc*) -> Simulink-PS Converter11/1
  Constant54/1 -> Encoder5/3(N)
  Low-Pass Filter Speed Ref5/2(y_prev_out) -> Unit Delay35/1
  Step10/1 -> Gain18/1
  Low-Pass Filter Speed5/2(y_prev_out) -> Unit Delay33/1
  Mjerenje kuta i brzine5/1(we) -> Rate Transition12/1
  Mjerenje struje6/1(Output) -> Rate Transition10/1
  Rate Transition10/1 -> Demux5/1
  Diskretni regulatori struje6/1(ud_ref) -> PWM inverter5/1(ud_ref)
  Constant59/1 -> Low-Pass Filter Speed Ref5/4(fc)
  Encoder5/3(q_angle) -> Unit Delay32/1
  Encoder5/1(theta_e) -> Scope42/1, Goto25/1, Scope36/1
  Constant55/1 -> Encoder5/4(dt)
  Manual Switch11/1 -> Scope37/1, Diskretni regulatori struje6/2(iq_ref)
  Unit Delay33/1 -> Low-Pass Filter Speed5/2(y_prev)
  Unit Delay37/1 -> Low-Pass Filter Speed Ref5/3(x_prev)
  Low-Pass Filter Speed Ref5/3(x_prev_out) -> Unit Delay37/1
  Low-Pass Filter Speed5/1(y) -> Scope41/1, Goto22/1
  From40/1 -> Mjerenje struje6/1(Input)
  Unit Delay32/1 -> Encoder5/2(angle_prev)
  Constant56/1 -> Encoder5/5(pole_pairs)
  Constant58/1 -> Low-Pass Filter Current5/5(TS)
  Low-Pass Filter Speed Ref5/1(y) -> Scope39/1, Diskretni regulator brzine6/1(w_ref)
  Demux5/1 -> Diskretni regulatori struje6/3(id_mj)
  Mjerenje momenta5/1(Output) -> Terminator10/1
  Demux5/3 -> Terminator9/1
  Encoder5/2(omega_e) -> Low-Pass Filter Speed5/1(x), Scope36/2
  Constant51/1 -> Low-Pass Filter Speed Ref5/5(TS)
  Low-Pass Filter Speed5/3(x_prev_out) -> Unit Delay36/1
  Mjerenje kuta i brzine5/2(theta_e) -> Scope42/2, Encoder5/1(angle)
  Unit Delay34/1 -> Low-Pass Filter Current5/2(y_prev)
  [n_backeuler_emulation] -> Scope7/2
  [n_tustin_emulation] -> Scope7/3
  [n_backeuler_direct] -> Scope7/4
  [n_tustin_direct] -> Scope7/5
  Step11/1 -> [i_ref], Manual Switch7/1
  [i_ref] -> Manual Switch4/1
  [i_ref] -> Manual Switch6/1
  [i_ref] -> Manual Switch2/1
  [i_disc_emu_back] -> Scope43/2  "i_disc_emu_back"
  [i_disc_emu_tustin] -> Scope43/3  "i_disc_emu_tustin"
  [i_direct_back] -> Scope43/4  "i_direct_back"
  [i_direct_tustin] -> Scope43/5  "i_direct_tustin"
  [n_backeuler_emulation] -> To Workspace4/1
  [n_tustin_emulation] -> To Workspace5/1
  [n_backeuler_direct] -> To Workspace6/1
  [n_tustin_direct] -> To Workspace7/1
  From46/1 -> To Workspace/1  "i_disc_emu_back"
  From47/1 -> To Workspace1/1  "i_disc_emu_tustin"
  From48/1 -> To Workspace2/1  "i_direct_back"
  From49/1 -> To Workspace3/1  "i_direct_tustin"
  From50/1 -> To Workspace8/1  "i_ref"
  [n_ref] -> To Workspace9/1
  connections:
  Solver Configuration6/RConn1 -- Controlled Voltage Source (Three-Phase)7/RConn1 -- Mjerenje struje5/LConn1
  Electrical Reference6/LConn1 -- Controlled Voltage Source (Three-Phase)7/LConn2
  PMSM7/RConn2 -- Mechanical Rotational Reference12/LConn1
  PMSM7/RConn1 -- Mjerenje momenta6/LConn1
  Simulink-PS Converter6/RConn1 -- Controlled Voltage Source (Three-Phase)7/LConn1
  Mjerenje struje5/RConn1 -- PMSM7/LConn1
  Simulink-PS Converter/RConn1 -- Ideal Torque Source7/RConn1
  Mjerenje kuta i brzine6/LConn1 -- Ideal Torque Source7/LConn1 -- Mjerenje momenta6/RConn1 -- Inertia/LConn1
  Mjerenje momenta3/RConn1 -- Inertia1/LConn1 -- Mjerenje kuta i brzine3/LConn1 -- Ideal Torque Source4/LConn1
  Mjerenje struje2/LConn1 -- Solver Configuration2/RConn1 -- Controlled Voltage Source (Three-Phase)4/RConn1
  Simulink-PS Converter7/RConn1 -- Controlled Voltage Source (Three-Phase)4/LConn1
  Electrical Reference3/LConn1 -- Controlled Voltage Source (Three-Phase)4/LConn2
  PMSM4/RConn1 -- Mjerenje momenta3/LConn1
  PMSM4/RConn2 -- Mechanical Rotational Reference6/LConn1
  Mjerenje struje2/RConn1 -- PMSM4/LConn1
  Simulink-PS Converter3/RConn1 -- Ideal Torque Source4/RConn1
  Mjerenje momenta2/RConn1 -- Inertia2/LConn1 -- Mjerenje kuta i brzine2/LConn1 -- Ideal Torque Source3/LConn1
  Mjerenje struje1/LConn1 -- Solver Configuration1/RConn1 -- Controlled Voltage Source (Three-Phase)3/RConn1
  Simulink-PS Converter1/RConn1 -- Ideal Torque Source3/RConn1
  PMSM3/RConn2 -- Mechanical Rotational Reference4/LConn1
  Electrical Reference2/LConn1 -- Controlled Voltage Source (Three-Phase)3/LConn2
  Mjerenje struje1/RConn1 -- PMSM3/LConn1
  Simulink-PS Converter5/RConn1 -- Controlled Voltage Source (Three-Phase)3/LConn1
  PMSM3/RConn1 -- Mjerenje momenta2/LConn1
  Mjerenje kuta i brzine1/LConn1 -- Inertia3/LConn1 -- Ideal Torque Source1/LConn1 -- Mjerenje momenta1/RConn1
  Mjerenje struje3/LConn1 -- Solver Configuration3/RConn1 -- Controlled Voltage Source (Three-Phase)1/RConn1
  Simulink-PS Converter2/RConn1 -- Ideal Torque Source1/RConn1
  Simulink-PS Converter4/RConn1 -- Controlled Voltage Source (Three-Phase)1/LConn1
  PMSM1/RConn1 -- Mjerenje momenta1/LConn1
  PMSM1/RConn2 -- Mechanical Rotational Reference3/LConn1
  Mjerenje struje3/RConn1 -- PMSM1/LConn1
  Electrical Reference1/LConn1 -- Controlled Voltage Source (Three-Phase)1/LConn2
  Mjerenje kuta i brzine4/LConn1 -- Inertia4/LConn1 -- Ideal Torque Source2/LConn1 -- Mjerenje momenta4/RConn1
  Mjerenje struje4/LConn1 -- Solver Configuration4/RConn1 -- Controlled Voltage Source (Three-Phase)2/RConn1
  Ideal Torque Source2/RConn2 -- Mechanical Rotational Reference7/LConn1
  Simulink-PS Converter8/RConn1 -- Ideal Torque Source2/RConn1
  Mjerenje struje4/RConn1 -- PMSM2/LConn1
  Simulink-PS Converter9/RConn1 -- Controlled Voltage Source (Three-Phase)2/LConn1
  PMSM2/RConn2 -- Mechanical Rotational Reference8/LConn1
  PMSM2/RConn1 -- Mjerenje momenta4/LConn1
  Electrical Reference4/LConn1 -- Controlled Voltage Source (Three-Phase)2/LConn2
  Mjerenje momenta5/RConn1 -- Ideal Torque Source5/LConn1 -- Mjerenje kuta i brzine5/LConn1 -- Inertia5/LConn1
  Controlled Voltage Source (Three-Phase)5/RConn1 -- Mjerenje struje6/LConn1 -- Solver Configuration5/RConn1
  PMSM5/RConn2 -- Mechanical Rotational Reference10/LConn1
  Simulink-PS Converter11/RConn1 -- Controlled Voltage Source (Three-Phase)5/LConn1
  Mjerenje struje6/RConn1 -- PMSM5/LConn1
  Ideal Torque Source5/RConn2 -- Mechanical Rotational Reference9/LConn1
  Electrical Reference5/LConn1 -- Controlled Voltage Source (Three-Phase)5/LConn2
  Simulink-PS Converter10/RConn1 -- Ideal Torque Source5/RConn1
  PMSM5/RConn1 -- Mjerenje momenta5/LConn1
  Ideal Torque Source4/RConn2 -- Mechanical Rotational Reference5/LConn1
  Ideal Torque Source1/RConn2 -- Mechanical Rotational Reference2/LConn1
  Ideal Torque Source3/RConn2 -- Mechanical Rotational Reference1/LConn1
  Ideal Torque Source7/RConn2 -- Mechanical Rotational Reference11/LConn1
